simulink model "TMS_20260330_1321"  (R2024b)
settings: Solver=VariableStepAuto  StartTime=0.0  StopTime=10.0  RelTol=1e-3
settings Model: Creator=uiv53217  LastModifiedBy=uiv53217

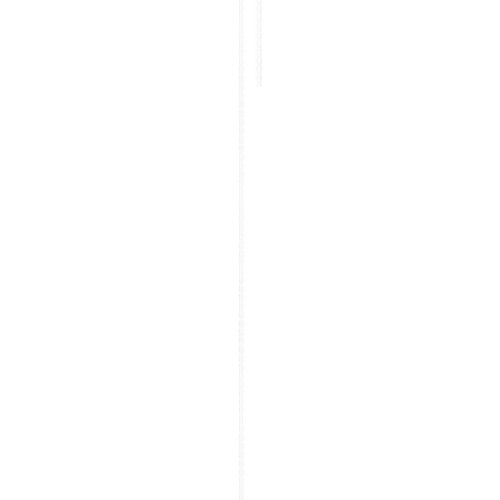
[thumbnail: Simulink's stored preview of the top-level diagram]
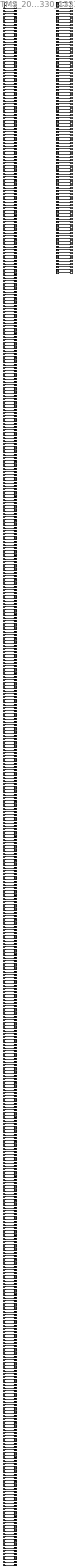
== system TMS_20260330_1321 ==
  OnOffReq_FL : Inport  OutDataTypeStr=uint8
  OnOffReq_FR : Inport  Port=2  OutDataTypeStr=uint8
  OnOffReq_RL : Inport  Port=3  OutDataTypeStr=uint8
  AutoReq_FL : Inport  Port=4  OutDataTypeStr=uint8
  AutoReq_FR : Inport  Port=5  OutDataTypeStr=uint8
  AutoReq_RL : Inport  Port=6  OutDataTypeStr=uint8
  MaxDefReq : Inport  Port=7  OutDataTypeStr=uint8
  FastVent : Inport  Port=8  OutDataTypeStr=uint8
  MaxACReq : Inport  Port=9  OutDataTypeStr=uint8
  MaxHeatReq : Inport  Port=10  OutDataTypeStr=uint8
  SmartClearReq : Inport  Port=11  OutDataTypeStr=uint8
  ACReq_FL : Inport  Port=12  OutDataTypeStr=uint8
  ACReq_FR : Inport  Port=13  OutDataTypeStr=uint8
  ACReq_RL : Inport  Port=14  OutDataTypeStr=uint8
  HeatReq_FL : Inport  Port=15  OutDataTypeStr=uint8
  HeatReq_FR : Inport  Port=16  OutDataTypeStr=uint8
  HeatReq_RL : Inport  Port=17  OutDataTypeStr=uint8
  VentReq_FL : Inport  Port=18  OutDataTypeStr=uint8
  VentReq_FR : Inport  Port=19  OutDataTypeStr=uint8
  VentReq_RL : Inport  Port=20  OutDataTypeStr=uint8
  TSet_FL : Inport  Port=21  OutDataTypeStr=uint16
  TSet_FR : Inport  Port=22  OutDataTypeStr=uint16
  TSet_RL : Inport  Port=23  OutDataTypeStr=uint16
  WindLvl_FL : Inport  Port=24  OutDataTypeStr=uint8
  WindLvl_FR : Inport  Port=25  OutDataTypeStr=uint8
  WindLvl_RL : Inport  Port=26  OutDataTypeStr=uint8
  OutletMode_FL : Inport  Port=27  OutDataTypeStr=uint8
  OutletMode_FR : Inport  Port=28  OutDataTypeStr=uint8
  OutletMode_RL : Inport  Port=29  OutDataTypeStr=uint8
  Sync : Inport  Port=30  OutDataTypeStr=uint8
  Inlet : Inport  Port=31  OutDataTypeStr=uint8
  ECO : Inport  Port=32  OutDataTypeStr=uint8
  AQS : Inport  Port=33  OutDataTypeStr=uint8
  RrWndHet : Inport  Port=34  OutDataTypeStr=uint8
  CfgAutoWindLvl : Inport  Port=35  OutDataTypeStr=uint8
  ACFrtPnlLckRrPnl : Inport  Port=36  OutDataTypeStr=uint8
  OccupantStsFL : Inport  Port=37  OutDataTypeStr=uint8
  OccupantStsFR : Inport  Port=38  OutDataTypeStr=uint8
  OccupantStsRL : Inport  Port=39  OutDataTypeStr=uint8
  OccupantStsRM : Inport  Port=40  OutDataTypeStr=uint8
  OccupantStsRR : Inport  Port=41  OutDataTypeStr=uint8
  CmptmtFrntWindDewT : Inport  Port=42  OutDataTypeStr=uint16
  CmptmtFrntWindT : Inport  Port=43  OutDataTypeStr=uint16
  CmptmtRelHum : Inport  Port=44  OutDataTypeStr=uint16
  RiSolarData : Inport  Port=45  OutDataTypeStr=uint8
  LeSolarData : Inport  Port=46  OutDataTypeStr=uint8
  VehSpd : Inport  Port=47  OutDataTypeStr=uint16
  CarModSts : Inport  Port=48  OutDataTypeStr=uint8
  UsgModSts : Inport  Port=49  OutDataTypeStr=uint8
  Cal_Sig_AmbTEna : Inport  Port=50  OutDataTypeStr=uint8
  Cal_Sig_AmbT : Inport  Port=51  OutDataTypeStr=uint16
  Cal_Sig_InCarTEna : Inport  Port=52  OutDataTypeStr=uint8
  Cal_Sig_InCarT : Inport  Port=53  OutDataTypeStr=uint16
  Cal_Sig_HvacEvaprTFrntEna : Inport  Port=54  OutDataTypeStr=uint8
  Cal_Sig_HvacEvaprTFrntT : Inport  Port=55  OutDataTypeStr=uint16
  Cal_Sig_HvacEvaprTReEna : Inport  Port=56  OutDataTypeStr=uint8
  Cal_Sig_HvacEvaprTReT : Inport  Port=57  OutDataTypeStr=uint16
  Cal_Sig_HvacCondsorTFrntTEna : Inport  Port=58  OutDataTypeStr=uint8
  Cal_Sig_HvacCondsorTFrntT : Inport  Port=59  OutDataTypeStr=uint16
  Cal_Sig_CooltT1Ena : Inport  Port=60  OutDataTypeStr=uint8
  Cal_Sig_CooltT1 : Inport  Port=61  OutDataTypeStr=uint16
  Cal_Sig_CooltT2Ena : Inport  Port=62  OutDataTypeStr=uint8
  Cal_Sig_CooltT2 : Inport  Port=63  OutDataTypeStr=uint16
  Cal_Sig_CooltT3Ena : Inport  Port=64  OutDataTypeStr=uint8
  Cal_Sig_CooltT3 : Inport  Port=65  OutDataTypeStr=uint16
  AutoDeHumPopUp : Inport  Port=66  OutDataTypeStr=uint8
  AutoDefrstPopUp : Inport  Port=67  OutDataTypeStr=uint8
  AutoFreshPopUp : Inport  Port=68  OutDataTypeStr=uint8
  ClimaDefrstSts : Inport  Port=69  OutDataTypeStr=uint8
  ClimaDefrstMaxSts : Inport  Port=70  OutDataTypeStr=uint8
  HvacFrntBlowerSts : Inport  Port=71  OutDataTypeStr=uint8
  HvacReBlowerSts : Inport  Port=72  OutDataTypeStr=uint8
  HvacAirMFlwFrntEstimd : Inport  Port=73  OutDataTypeStr=uint16
  HvacAirMFlwReEstimd : Inport  Port=74  OutDataTypeStr=uint16
  HvacAirQFlwFrntEstimd : Inport  Port=75  OutDataTypeStr=uint16
  HvacAirQFlwReEstimd : Inport  Port=76  OutDataTypeStr=uint16
  HvacFrntBlwSpdFb : Inport  Port=77  OutDataTypeStr=uint16
  HvacReBlwSpdFb : Inport  Port=78  OutDataTypeStr=uint16
  HvacCoolgEnaFrnt : Inport  Port=79  OutDataTypeStr=uint8
  HvacCoolgEnaRe : Inport  Port=80  OutDataTypeStr=uint8
  HvacDefrstFlapActlPosn : Inport  Port=81  OutDataTypeStr=uint16
  HvacEvaprTSpFrnt : Inport  Port=82  OutDataTypeStr=uint16
  HvacEvaprTSpRe : Inport  Port=83  OutDataTypeStr=uint16
  HvacModFlapActlPosnFrstRowLe : Inport  Port=84  OutDataTypeStr=uint16
  HvacModFlapActlPosnFrstRowRi : Inport  Port=85  OutDataTypeStr=uint16
  HvacModFlapActlPosnSecRowLe : Inport  Port=86  OutDataTypeStr=uint16
  HvacModFlapActlPosnSecRowRi : Inport  Port=87  OutDataTypeStr=uint16
  HvacOsaFlapActlPosn : Inport  Port=88  OutDataTypeStr=uint16
  HvacRecFlapActlPosn : Inport  Port=89  OutDataTypeStr=uint16
  HvacRecircActRat : Inport  Port=90  OutDataTypeStr=uint8
  HvacTempFlapActlPosnFrstRowLe : Inport  Port=91  OutDataTypeStr=uint16
  HvacTempFlapActlPosnFrstRowRi : Inport  Port=92  OutDataTypeStr=uint16
  HvacTempFlapActlPosnSecRowLe : Inport  Port=93  OutDataTypeStr=uint16
  HvacTempFlapActlPosnSecRowRi : Inport  Port=94  OutDataTypeStr=uint16
  HvacTgtAirTForRowFirstLe : Inport  Port=95  OutDataTypeStr=uint16
  HvacTgtAirTForRowFirstRi : Inport  Port=96  OutDataTypeStr=uint16
  HvacTgtAirTForRowSecLe : Inport  Port=97  OutDataTypeStr=uint16
  HvacTgtAirTForRowSecRi : Inport  Port=98  OutDataTypeStr=uint16
  AmbTEstimdAmbTEstimd : Inport  Port=99  OutDataTypeStr=uint16
  AmbTEstimdQf : Inport  Port=100  OutDataTypeStr=uint8
  CmptmtTFrntCmptmtTFrnt : Inport  Port=101  OutDataTypeStr=uint16
  CmptmtTFrntFanForCmptmtTRunng : Inport  Port=102  OutDataTypeStr=uint8
  CmptmtTFrntQf : Inport  Port=103  OutDataTypeStr=uint8
  CmptmtTReCmptmtTFrnt : Inport  Port=104  OutDataTypeStr=uint16
  CmptmtTReCmptmtTFrntQf : Inport  Port=105  OutDataTypeStr=uint8
  CmptmtTReFanForCmptmtTRunng : Inport  Port=106  OutDataTypeStr=uint8
  HvacEvaprTFrntTHvac : Inport  Port=107  OutDataTypeStr=uint16
  HvacEvaprTFrntTQf : Inport  Port=108  OutDataTypeStr=uint8
  HvacEvaprTReTHvac : Inport  Port=109  OutDataTypeStr=uint16
  HvacEvaprTReTQf : Inport  Port=110  OutDataTypeStr=uint8
  HvacAirTForRowFirstAtFlrLeTHvac : Inport  Port=111  OutDataTypeStr=uint16
  HvacAirTForRowFirstAtFlrLeTQf : Inport  Port=112  OutDataTypeStr=uint8
  HvacAirTForRowFirstAtFlrRiTHvac : Inport  Port=113  OutDataTypeStr=uint16
  HvacAirTForRowFirstAtFlrRiTQf : Inport  Port=114  OutDataTypeStr=uint8
  HvacAirTForRowFirstAtFaceLeTHvac : Inport  Port=115  OutDataTypeStr=uint16
  HvacAirTForRowFirstAtFaceLeTQf : Inport  Port=116  OutDataTypeStr=uint8
  HvacAirTForRowFirstAtFaceRiTHvac : Inport  Port=117  OutDataTypeStr=uint16
  HvacAirTForRowFirstAtFaceRiTQf : Inport  Port=118  OutDataTypeStr=uint8
  HvacAirTForRowSecAtFlrLeTHvac : Inport  Port=119  OutDataTypeStr=uint16
  HvacAirTForRowSecAtFlrLeTQf : Inport  Port=120  OutDataTypeStr=uint8
  HvacAirTForRowSecAtFlrRiTHvac : Inport  Port=121  OutDataTypeStr=uint16
  HvacAirTForRowSecAtFlrRiTQf : Inport  Port=122  OutDataTypeStr=uint8
  HvacAirTForRowSecAtFaceLeTHvac : Inport  Port=123  OutDataTypeStr=uint16
  HvacAirTForRowSecAtFaceLeTQf : Inport  Port=124  OutDataTypeStr=uint8
  HvacAirTForRowSecAtFaceRiTHvac : Inport  Port=125  OutDataTypeStr=uint16
  HvacAirTForRowSecAtFaceRiTQf : Inport  Port=126  OutDataTypeStr=uint8
  HvacCondsorTFrntTHvac : Inport  Port=127  OutDataTypeStr=uint16
  HvacCondsorTFrntTQf : Inport  Port=128  OutDataTypeStr=uint8
  HvacCondsorTspFrntTHvac : Inport  Port=129  OutDataTypeStr=uint16
  ClimaThermReq : Inport  Port=130  OutDataTypeStr=uint8
  ClimaThermSts : Inport  Port=131  OutDataTypeStr=uint8
  HvacAirTHvacIntkT : Inport  Port=132  OutDataTypeStr=uint16
  RsvdSigForClima01 : Inport  Port=133  OutDataTypeStr=uint8
  RsvdSigForClima02 : Inport  Port=134  OutDataTypeStr=uint8
  RsvdSigForClima03 : Inport  Port=135  OutDataTypeStr=uint8
  RsvdSigForClima04 : Inport  Port=136  OutDataTypeStr=uint8
  RsvdSigForClima05 : Inport  Port=137  OutDataTypeStr=uint8
  RsvdSigForClima06 : Inport  Port=138  OutDataTypeStr=uint8
  RsvdSigForClima07 : Inport  Port=139  OutDataTypeStr=uint8
  RsvdSigForClima08 : Inport  Port=140  OutDataTypeStr=uint8
  RsvdSigForClima09 : Inport  Port=141  OutDataTypeStr=uint8
  RsvdSigForClima10 : Inport  Port=142  OutDataTypeStr=uint8
  RsvdSigForClima11 : Inport  Port=143  OutDataTypeStr=uint8
  RsvdSigForClima12 : Inport  Port=144  OutDataTypeStr=uint8
  RsvdSigForClima13 : Inport  Port=145  OutDataTypeStr=uint8
  RsvdSigForClima14 : Inport  Port=146  OutDataTypeStr=uint8
  RsvdSigForClima15 : Inport  Port=147  OutDataTypeStr=uint8
  RsvdSigForClima16 : Inport  Port=148  OutDataTypeStr=uint8
  RsvdSigForClima17 : Inport  Port=149  OutDataTypeStr=uint8
  RsvdSigForClima18 : Inport  Port=150  OutDataTypeStr=uint8
  RsvdSigForClima19 : Inport  Port=151  OutDataTypeStr=uint8
  RsvdSigForClima20 : Inport  Port=152  OutDataTypeStr=uint8
  RsvdSigForClima21 : Inport  Port=153  OutDataTypeStr=uint8
  RsvdSigForClima22 : Inport  Port=154  OutDataTypeStr=uint8
  RsvdSigForClima23 : Inport  Port=155  OutDataTypeStr=uint8
  HvacDefrstFlapTgtPosn : Inport  Port=156  OutDataTypeStr=uint16
  HvacModFlapTgtPosnFrstRowLe : Inport  Port=157  OutDataTypeStr=uint16
  HvacModFlapTgtPosnFrstRowRi : Inport  Port=158  OutDataTypeStr=uint16
  HvacModFlapTgtPosnSecRowLe : Inport  Port=159  OutDataTypeStr=uint16
  HvacModFlapTgtPosnSecRowRi : Inport  Port=160  OutDataTypeStr=uint16
  HvacOsaFlapTgtPosn : Inport  Port=161  OutDataTypeStr=uint16
  HvacRecFlapTgtPosn : Inport  Port=162  OutDataTypeStr=uint16
  HvacTempFlapTgtPosnFrstRowLe : Inport  Port=163  OutDataTypeStr=uint16
  HvacTempFlapTgtPosnFrstRowRi : Inport  Port=164  OutDataTypeStr=uint16
  HvacTempFlapTgtPosnSecRowLe : Inport  Port=165  OutDataTypeStr=uint16
  HvacTempFlapTgtPosnSecRowRi : Inport  Port=166  OutDataTypeStr=uint16
  HvBattThermRunAway : Inport  Port=167  OutDataTypeStr=uint8
  WhlMotCooltFlowMinReq : Inport  Port=168  OutDataTypeStr=uint16
  WhlMotSysCoolgReq : Inport  Port=169  OutDataTypeStr=uint8
  WhlMotSysCooltT : Inport  Port=170  OutDataTypeStr=uint16
  WhlMotSysInvrT : Inport  Port=171  OutDataTypeStr=uint16
  WhlMotSysMotT : Inport  Port=172  OutDataTypeStr=uint16
  DCChrgSt : Inport  Port=173  OutDataTypeStr=uint8
  DCChrgnHndlSts : Inport  Port=174  OutDataTypeStr=uint8
  ACChrgSt : Inport  Port=175  OutDataTypeStr=uint8
  ACChrgnHndlSts : Inport  Port=176  OutDataTypeStr=uint8
  HvBattCooltFlowReq : Inport  Port=177  OutDataTypeStr=uint16
  HvBattCooltMaxTReq : Inport  Port=178  OutDataTypeStr=uint16
  HvBattCooltMinTReq : Inport  Port=179  OutDataTypeStr=uint16
  HvBattCooltTReq : Inport  Port=180  OutDataTypeStr=uint16
  HvBattThermReq : Inport  Port=181  OutDataTypeStr=uint8
  HvBattTAvg : Inport  Port=182  OutDataTypeStr=uint16
  HvBattTMax : Inport  Port=183  OutDataTypeStr=uint16
  HvBattTMin : Inport  Port=184  OutDataTypeStr=uint16
  HvBattActSOC : Inport  Port=185  OutDataTypeStr=uint16
  HvSysRlyStsChks : Inport  Port=186  OutDataTypeStr=uint8
  HvSysRlyStsCntr : Inport  Port=187  OutDataTypeStr=uint8
  HvSysRlyStsHvSysRlySts : Inport  Port=188  OutDataTypeStr=uint8
  HvCmprPwrAllwd : Inport  Port=189  OutDataTypeStr=uint8
  HvHeatrPwrAllwd : Inport  Port=190  OutDataTypeStr=uint8
  WhlMotCooltFlwEstimd : Inport  Port=191  OutDataTypeStr=uint16
  HvBattCooltFlwEstimd : Inport  Port=192  OutDataTypeStr=uint16
  HvBattThermReqFb : Inport  Port=193  OutDataTypeStr=uint8
  HvCmprNormPwrDes : Inport  Port=194  OutDataTypeStr=uint8
  HvHeatrNormPwrDes : Inport  Port=195  OutDataTypeStr=uint8
  HvCmprCritPwrDes : Inport  Port=196  OutDataTypeStr=uint8
  HvHeatrCritPwrDes : Inport  Port=197  OutDataTypeStr=uint8
  ThermDeiceReq : Inport  Port=198  OutDataTypeStr=uint8
  ThermRfgModReq : Inport  Port=199  OutDataTypeStr=uint8
  ThermRfgModSts : Inport  Port=200  OutDataTypeStr=uint8
  ThermRfgModSwtSts : Inport  Port=201  OutDataTypeStr=uint8
  ThermCooltModReq : Inport  Port=202  OutDataTypeStr=uint8
  ThermCooltModSts : Inport  Port=203  OutDataTypeStr=uint8
  ThermCooltModSwtSts : Inport  Port=204  OutDataTypeStr=uint8
  RfgSnsrT1 : Inport  Port=205  OutDataTypeStr=uint16
  RfgSnsrT2 : Inport  Port=206  OutDataTypeStr=uint16
  RfgSnsrT3 : Inport  Port=207  OutDataTypeStr=uint16
  RfgSnsrT4 : Inport  Port=208  OutDataTypeStr=uint16
  RfgSnsrP1 : Inport  Port=209  OutDataTypeStr=uint16
  RfgSnsrPT1T : Inport  Port=210  OutDataTypeStr=uint16
  RfgSnsrPT1P : Inport  Port=211  OutDataTypeStr=uint16
  RfgSnsrT5Rsvd : Inport  Port=212  OutDataTypeStr=uint16
  RfgSnsrT6Rsvd : Inport  Port=213  OutDataTypeStr=uint16
  RfgSnsrT7Rsvd : Inport  Port=214  OutDataTypeStr=uint16
  RfgSnsrT8Rsvd : Inport  Port=215  OutDataTypeStr=uint16
  RfgSnsrP5Rsvd : Inport  Port=216  OutDataTypeStr=uint16
  RfgSnsrP6Rsvd : Inport  Port=217  OutDataTypeStr=uint16
  RfgSnsrP7Rsvd : Inport  Port=218  OutDataTypeStr=uint16
  RfgSnsrP8Rsvd : Inport  Port=219  OutDataTypeStr=uint16
  CooltSnsrT1 : Inport  Port=220  OutDataTypeStr=uint16
  CooltSnsrT2 : Inport  Port=221  OutDataTypeStr=uint16
  CooltSnsrT3 : Inport  Port=222  OutDataTypeStr=uint16
  CooltSnsrT4Rsvd : Inport  Port=223  OutDataTypeStr=uint16
  CooltSnsrT5Rsvd : Inport  Port=224  OutDataTypeStr=uint16
  CooltSnsrT6Rsvd : Inport  Port=225  OutDataTypeStr=uint16
  CooltSnsrT7Rsvd : Inport  Port=226  OutDataTypeStr=uint16
  CooltSnsrT8Rsvd : Inport  Port=227  OutDataTypeStr=uint16
  CRFMAirMFlwEstimd : Inport  Port=228  OutDataTypeStr=uint16
  CRFMAirQFlwEstimd : Inport  Port=229  OutDataTypeStr=uint16
  ThermCptsSts : Inport  Port=230  OutDataTypeStr=uint32
  ThermProtnSts : Inport  Port=231  OutDataTypeStr=uint32
  ThermSysSts : Inport  Port=232  OutDataTypeStr=uint8
  RsvdSigForTherm01 : Inport  Port=233  OutDataTypeStr=uint8
  RsvdSigForTherm02 : Inport  Port=234  OutDataTypeStr=uint8
  RsvdSigForTherm03 : Inport  Port=235  OutDataTypeStr=uint8
  RsvdSigForTherm04 : Inport  Port=236  OutDataTypeStr=uint8
  RsvdSigForTherm05 : Inport  Port=237  OutDataTypeStr=uint8
  RsvdSigForTherm06 : Inport  Port=238  OutDataTypeStr=uint8
  RsvdSigForTherm07 : Inport  Port=239  OutDataTypeStr=uint8
  RsvdSigForTherm08 : Inport  Port=240  OutDataTypeStr=uint8
  RsvdSigForTherm09 : Inport  Port=241  OutDataTypeStr=uint8
  RsvdSigForTherm10 : Inport  Port=242  OutDataTypeStr=uint8
  RsvdSigForTherm11 : Inport  Port=243  OutDataTypeStr=uint8
  RsvdSigForTherm12 : Inport  Port=244  OutDataTypeStr=uint8
  RsvdSigForTherm13 : Inport  Port=245  OutDataTypeStr=uint8
  RsvdSigForTherm14 : Inport  Port=246  OutDataTypeStr=uint8
  RsvdSigForTherm15 : Inport  Port=247  OutDataTypeStr=uint8
  RsvdSigForTherm16 : Inport  Port=248  OutDataTypeStr=uint8
  RsvdSigForTherm17 : Inport  Port=249  OutDataTypeStr=uint8
  RsvdSigForTherm18 : Inport  Port=250  OutDataTypeStr=uint8
  RsvdSigForTherm19 : Inport  Port=251  OutDataTypeStr=uint8
  RsvdSigForTherm20 : Inport  Port=252  OutDataTypeStr=uint8
  RsvdSigForTherm21 : Inport  Port=253  OutDataTypeStr=uint8
  RsvdSigForTherm22 : Inport  Port=254  OutDataTypeStr=uint8
  RsvdSigForTherm23 : Inport  Port=255  OutDataTypeStr=uint8
  HeatrPmpPwmCmd : Inport  Port=256  OutDataTypeStr=uint16
  HvBattPmpPwmCmd : Inport  Port=257  OutDataTypeStr=uint16
  EldtPmpPwmCmd : Inport  Port=258  OutDataTypeStr=uint16
  SOV1OnOffCmd : Inport  Port=259  OutDataTypeStr=uint8
  SOV2OnOffCmd : Inport  Port=260  OutDataTypeStr=uint8
  SOV3OnOffCmd : Inport  Port=261  OutDataTypeStr=uint8
  CoolgFanPWMCmd : Inport  Port=262  OutDataTypeStr=uint16
  FrntBlwPWMCmd : Inport  Port=263  OutDataTypeStr=uint16
  BcfvNVMFlt : Inport  Port=264  OutDataTypeStr=uint8
  BctvNVMFlt : Inport  Port=265  OutDataTypeStr=uint8
  CmprEEPROMFault : Inport  Port=266  OutDataTypeStr=uint8
  CmprHVoltResonanceStat : Inport  Port=267  OutDataTypeStr=uint8
  CmprInCurrOverCurrStat : Inport  Port=268  OutDataTypeStr=uint8
  CmprLiquidSluggingStat : Inport  Port=269  OutDataTypeStr=uint8
  CmprLostCommStat : Inport  Port=270  OutDataTypeStr=uint8
  CmprMotorCurrOverCurrStat : Inport  Port=271  OutDataTypeStr=uint8
  CmprOverMotorCurrStat : Inport  Port=272  OutDataTypeStr=uint8
  CmprOverPowerStat : Inport  Port=273  OutDataTypeStr=uint8
  CmprRAMFault : Inport  Port=274  OutDataTypeStr=uint8
  CmprROMFault : Inport  Port=275  OutDataTypeStr=uint8
  CmprReqCmprPwrLim : Inport  Port=276  OutDataTypeStr=uint8
  CmprReqCmprRunReq : Inport  Port=277  OutDataTypeStr=uint8
  CmprReqCmprSpdReq : Inport  Port=278  OutDataTypeStr=uint8
  CmprRotorLockStat : Inport  Port=279  OutDataTypeStr=uint8
  CmprSpdIncrReq : Inport  Port=280  OutDataTypeStr=uint8
  CooltFlowInCmptmtCirc : Inport  Port=281  OutDataTypeStr=uint16
  HpBattFwvActvSaveReq : Inport  Port=282  OutDataTypeStr=uint8
  HpBattFwvFltSts : Inport  Port=283  OutDataTypeStr=uint8
  HpBattFwvMode : Inport  Port=284  OutDataTypeStr=uint8
  HpBattFwvPosRec : Inport  Port=285  OutDataTypeStr=uint16
  HpBattFwvPosSetReq : Inport  Port=286  OutDataTypeStr=uint8
  HpBattFwvRefDrvReq : Inport  Port=287  OutDataTypeStr=uint8
  HpBattFwvRunSts : Inport  Port=288  OutDataTypeStr=uint8
  HpBattFwvSpdLvl : Inport  Port=289  OutDataTypeStr=uint8
  HpBattFwvSpdLvlReq : Inport  Port=290  OutDataTypeStr=uint8
  HpBattFwvTempSts : Inport  Port=291  OutDataTypeStr=uint8
  HpBattFwvVoltSts : Inport  Port=292  OutDataTypeStr=uint8
  HpBattVlvActvSaveReq : Inport  Port=293  OutDataTypeStr=uint8
  HpBattVlvFltSts : Inport  Port=294  OutDataTypeStr=uint8
  HpBattVlvMode : Inport  Port=295  OutDataTypeStr=uint8
  HpBattVlvPosRec : Inport  Port=296  OutDataTypeStr=uint16
  HpBattVlvPosSetReq : Inport  Port=297  OutDataTypeStr=uint8
  HpBattVlvRefDrvReq : Inport  Port=298  OutDataTypeStr=uint8
  HpBattVlvRunSts : Inport  Port=299  OutDataTypeStr=uint8
  HpBattVlvSpdLvl : Inport  Port=300  OutDataTypeStr=uint8
  HpBattVlvSpdLvlReq : Inport  Port=301  OutDataTypeStr=uint8
  HpBattVlvTempSts : Inport  Port=302  OutDataTypeStr=uint8
  HpBattVlvVoltSts : Inport  Port=303  OutDataTypeStr=uint8
  HvCooltHeatrEnad : Inport  Port=304  OutDataTypeStr=uint8
  HvCooltHeatrICnsSig : Inport  Port=305  OutDataTypeStr=uint8
  HvCooltHeatrInfoCompProtn : Inport  Port=306  OutDataTypeStr=uint8
  HvCooltHeatrSplyUForCtrlUnitValSig : Inport  Port=307  OutDataTypeStr=uint8
  HvCooltHeatrStsSig : Inport  Port=308  OutDataTypeStr=uint8
  HvCooltWtrHeatrWtrTInIntk : Inport  Port=309  OutDataTypeStr=uint8
  HvCooltWtrHeatrWtrTInOutl : Inport  Port=310  OutDataTypeStr=uint8
  HvHeatrPwrCns : Inport  Port=311  OutDataTypeStr=uint16
  HvHeatrPwrCnsDes : Inport  Port=312  OutDataTypeStr=uint16
  HvWtrHeatrPwrCnsAllwd : Inport  Port=313  OutDataTypeStr=uint8
  HvWtrHeatrWtrTDes : Inport  Port=314  OutDataTypeStr=uint8
  CmprDiagcFbCmprCmprSpdErr : Inport  Port=315  OutDataTypeStr=uint8
  CmprDiagcFbCmprCtrlrErr : Inport  Port=316  OutDataTypeStr=uint8
  CmprDiagcFbCmprDrvrCircSnsr : Inport  Port=317  OutDataTypeStr=uint8
  CmprDiagcFbCmprDrvrCircSnsrPlaus : Inport  Port=318  OutDataTypeStr=uint8
  CmprDiagcFbCmprHvSnsr1 : Inport  Port=319  OutDataTypeStr=uint8
  CmprDiagcFbCmprHvSnsr2 : Inport  Port=320  OutDataTypeStr=uint8
  CmprDiagcFbCmprHvSnsrI : Inport  Port=321  OutDataTypeStr=uint8
  CmprDiagcFbCmprHvSnsrICrct : Inport  Port=322  OutDataTypeStr=uint8
  CmprDiagcFbCmprHvSnsrIPlaus : Inport  Port=323  OutDataTypeStr=uint8
  CmprDiagcFbCmprHvSnsrPlaus : Inport  Port=324  OutDataTypeStr=uint8
  CmprDiagcFbCmprHvSplyErr : Inport  Port=325  OutDataTypeStr=uint8
  CmprDiagcFbCmprPhaseWire : Inport  Port=326  OutDataTypeStr=uint8
  CmprDiagcFbCmprT1 : Inport  Port=327  OutDataTypeStr=uint8
  CmprDiagcFbCmprT2 : Inport  Port=328  OutDataTypeStr=uint8
  CmprDiagcFbCmprTOperErr1 : Inport  Port=329  OutDataTypeStr=uint8
  CmprDiagcFbCmprTOperErr2 : Inport  Port=330  OutDataTypeStr=uint8
  CmprDiagcFbCmprTPlaus : Inport  Port=331  OutDataTypeStr=uint8
  CmprDiagcFbCmprUSplyErr : Inport  Port=332  OutDataTypeStr=uint8
  CmprFbCmprI : Inport  Port=333  OutDataTypeStr=uint16
  CmprFbCmprIPha : Inport  Port=334  OutDataTypeStr=uint8
  CmprFbCmprSpd : Inport  Port=335  OutDataTypeStr=uint8
  CmprFbCmprSts1 : Inport  Port=336  OutDataTypeStr=uint8
  CmprFbCmprSts2 : Inport  Port=337  OutDataTypeStr=uint8
  CmprFbCmprT1 : Inport  Port=338  OutDataTypeStr=uint8
  CmprFbCmprT2 : Inport  Port=339  OutDataTypeStr=uint8
  CmprFbCmprU : Inport  Port=340  OutDataTypeStr=uint16
  EctvCmdVlvMovEna : Inport  Port=341  OutDataTypeStr=uint8
  EctvCmdVlvPosSetReq : Inport  Port=342  OutDataTypeStr=uint8
  EctvCmdVlvSpdLvlReq : Inport  Port=343  OutDataTypeStr=uint8
  EctvStatVlvFaultSts : Inport  Port=344  OutDataTypeStr=uint8
  EctvStatVlvPosSts : Inport  Port=345  OutDataTypeStr=uint8
  EctvStatVlvRunSts : Inport  Port=346  OutDataTypeStr=uint8
  EctvStatVlvSpdLvl : Inport  Port=347  OutDataTypeStr=uint8
  EctvStatVlvTempSts : Inport  Port=348  OutDataTypeStr=uint8
  EctvStatVoltSts : Inport  Port=349  OutDataTypeStr=uint8
  HvCooltHeatrEnadWhE2EChks : Inport  Port=350  OutDataTypeStr=uint8
  HvCooltHeatrEnadWhE2ECntr : Inport  Port=351  OutDataTypeStr=uint8
  HvCooltHeatrEnadWhE2EHvchEnad : Inport  Port=352  OutDataTypeStr=uint8
  HvCooltHeatrProtnOfSelfTmpSigHwProtn : Inport  Port=353  OutDataTypeStr=uint8
  HvCooltHeatrProtnOfSelfTmpSigOvrheatg : Inport  Port=354  OutDataTypeStr=uint8
  HvCooltHeatrProtnOfSelfTmpSigProtnOfSelfTmp : Inport  Port=355  OutDataTypeStr=uint8
  HvCooltHeatrProtnOfSelfTmpSigProtnOfSelfTmpResd : Inport  Port=356  OutDataTypeStr=uint8
  HvCooltHeatrSnsrFltSigCooltTInSnsrFlt : Inport  Port=357  OutDataTypeStr=uint8
  HvCooltHeatrSnsrFltSigCooltTOutSnsrFlt : Inport  Port=358  OutDataTypeStr=uint8
  HvCooltHeatrSnsrFltSigResdForSnsrFlt : Inport  Port=359  OutDataTypeStr=uint8
  HvCooltHeatrSnsrFltSigTInMtrlSnsrFlt : Inport  Port=360  OutDataTypeStr=uint8
  HvCooltHeatrSrvRqrdSigCircForDrvrShoOrOpen : Inport  Port=361  OutDataTypeStr=uint8
  HvCooltHeatrSrvRqrdSigICnsOutOfRng : Inport  Port=362  OutDataTypeStr=uint8
  HvCooltHeatrSrvRqrdSigMemErr : Inport  Port=363  OutDataTypeStr=uint8
  HvCooltHeatrSrvRqrdSigSrvRqrd : Inport  Port=364  OutDataTypeStr=uint8
  HvCooltHeatrSrvRqrdSigSrvRqrdResd : Inport  Port=365  OutDataTypeStr=uint8
  HvCooltHeatrStsWhE2EChks : Inport  Port=366  OutDataTypeStr=uint8
  HvCooltHeatrStsWhE2ECntr : Inport  Port=367  OutDataTypeStr=uint8
  HvCooltHeatrStsWhE2EHvchSts : Inport  Port=368  OutDataTypeStr=uint8
  HvCooltHeatrWarnSigCooltTOutOfRng : Inport  Port=369  OutDataTypeStr=uint8
  HvCooltHeatrWarnSigFltInCom : Inport  Port=370  OutDataTypeStr=uint8
  HvCooltHeatrWarnSigFltPrsnt : Inport  Port=371  OutDataTypeStr=uint8
  HvCooltHeatrWarnSigFltPrsntResd : Inport  Port=372  OutDataTypeStr=uint8
  HvCooltHeatrWarnSigHvOutOfRng : Inport  Port=373  OutDataTypeStr=uint8
  HvCooltHeatrWarnSigULoOutOfRng : Inport  Port=374  OutDataTypeStr=uint8
  BexvNVMFlt : Inport  Port=375  OutDataTypeStr=uint8
  CexvNVMFlt : Inport  Port=376  OutDataTypeStr=uint8
  EexvNVMFlt : Inport  Port=377  OutDataTypeStr=uint8
  BexvPosnReqExvCalibReq : Inport  Port=378  OutDataTypeStr=uint8
  BexvPosnReqExvHeatdReq : Inport  Port=379  OutDataTypeStr=uint8
  BexvPosnReqExvMovEnable : Inport  Port=380  OutDataTypeStr=uint8
  BexvPosnReqExvPosnReq : Inport  Port=381  OutDataTypeStr=uint16
  BexvStsExvActrPosn : Inport  Port=382  OutDataTypeStr=uint16
  BexvStsExvBlkErr : Inport  Port=383  OutDataTypeStr=uint8
  BexvStsExvCalibSts : Inport  Port=384  OutDataTypeStr=uint8
  BexvStsExvElecStsErr : Inport  Port=385  OutDataTypeStr=uint8
  BexvStsExvMovSts : Inport  Port=386  OutDataTypeStr=uint8
  BexvStsExvOvrTempErr : Inport  Port=387  OutDataTypeStr=uint8
  BexvStsExvOvrTrvlErr : Inport  Port=388  OutDataTypeStr=uint8
  BexvStsExvPreHeatgSts : Inport  Port=389  OutDataTypeStr=uint8
  BexvStsExvVoltgRangErr : Inport  Port=390  OutDataTypeStr=uint8
  CexvPosnReqExvCalibReq : Inport  Port=391  OutDataTypeStr=uint8
  CexvPosnReqExvHeatdReq : Inport  Port=392  OutDataTypeStr=uint8
  CexvPosnReqExvMovEnable : Inport  Port=393  OutDataTypeStr=uint8
  CexvPosnReqExvPosnReq : Inport  Port=394  OutDataTypeStr=uint16
  CexvStsExvActrPosn : Inport  Port=395  OutDataTypeStr=uint16
  CexvStsExvBlkErr : Inport  Port=396  OutDataTypeStr=uint8
  CexvStsExvCalibSts : Inport  Port=397  OutDataTypeStr=uint8
  CexvStsExvElecStsErr : Inport  Port=398  OutDataTypeStr=uint8
  CexvStsExvMovSts : Inport  Port=399  OutDataTypeStr=uint8
  CexvStsExvOvrTempErr : Inport  Port=400  OutDataTypeStr=uint8
  CexvStsExvOvrTrvlErr : Inport  Port=401  OutDataTypeStr=uint8
  CexvStsExvPreHeatgSts : Inport  Port=402  OutDataTypeStr=uint8
  CexvStsExvVoltgRangErr : Inport  Port=403  OutDataTypeStr=uint8
  EexvPosnReqExvCalibReq : Inport  Port=404  OutDataTypeStr=uint8
  EexvPosnReqExvHeatdReq : Inport  Port=405  OutDataTypeStr=uint8
  EexvPosnReqExvMovEnable : Inport  Port=406  OutDataTypeStr=uint8
  EexvPosnReqExvPosnReq : Inport  Port=407  OutDataTypeStr=uint16
  EexvStsExvActrPosn : Inport  Port=408  OutDataTypeStr=uint16
  EexvStsExvBlkErr : Inport  Port=409  OutDataTypeStr=uint8
  EexvStsExvCalibSts : Inport  Port=410  OutDataTypeStr=uint8
  EexvStsExvElecStsErr : Inport  Port=411  OutDataTypeStr=uint8
  EexvStsExvMovSts : Inport  Port=412  OutDataTypeStr=uint8
  EexvStsExvOvrTempErr : Inport  Port=413  OutDataTypeStr=uint8
  EexvStsExvOvrTrvlErr : Inport  Port=414  OutDataTypeStr=uint8
  EexvStsExvPreHeatgSts : Inport  Port=415  OutDataTypeStr=uint8
  EexvStsExvVoltgRangErr : Inport  Port=416  OutDataTypeStr=uint8
  AGMNVMFlt : Inport  Port=417  OutDataTypeStr=uint8
  GrlActTrqBoost : Inport  Port=418  OutDataTypeStr=uint8
  GrlAutoCalibReq : Inport  Port=419  OutDataTypeStr=uint8
  GrlHldTrqActive : Inport  Port=420  OutDataTypeStr=uint8
  GrlShttrMoveActive : Inport  Port=421  OutDataTypeStr=uint8
  GrlShttrOverVolt : Inport  Port=422  OutDataTypeStr=uint8
  GrlShttrOvertravelErr : Inport  Port=423  OutDataTypeStr=uint8
  GrlTrqBoostReq : Inport  Port=424  OutDataTypeStr=uint8
  GrlShttrDmdShttrCalEna : Inport  Port=425  OutDataTypeStr=uint8
  GrlShttrDmdShttrPosnReq : Inport  Port=426  OutDataTypeStr=uint8
  GrlShttrStsShttrActrFlt : Inport  Port=427  OutDataTypeStr=uint8
  GrlShttrStsShttrBlkd : Inport  Port=428  OutDataTypeStr=uint8
  GrlShttrStsShttrCalActv : Inport  Port=429  OutDataTypeStr=uint8
  GrlShttrStsShttrCalIndcd : Inport  Port=430  OutDataTypeStr=uint8
  GrlShttrStsShttrElecErr : Inport  Port=431  OutDataTypeStr=uint8
  GrlShttrStsShttrPosnRaw : Inport  Port=432  OutDataTypeStr=uint8
  GrlShttrStsShttrSnsrFlt : Inport  Port=433  OutDataTypeStr=uint8
  GrlShttrStsShttrTErr : Inport  Port=434  OutDataTypeStr=uint8
  GrlShttrStsShttrULoErr : Inport  Port=435  OutDataTypeStr=uint8
  AFUGenErr : Inport  Port=436  OutDataTypeStr=uint8
  AirFragActEnad : Inport  Port=437  OutDataTypeStr=uint8
  AirFragCh1 : Inport  Port=438  OutDataTypeStr=uint8
  AirFragCh1AvlTi : Inport  Port=439  OutDataTypeStr=uint16
  AirFragCh1RunngSts : Inport  Port=440  OutDataTypeStr=uint8
  AirFragCh1Type : Inport  Port=441  OutDataTypeStr=uint8
  AirFragCh2 : Inport  Port=442  OutDataTypeStr=uint8
  AirFragCh2AvlTi : Inport  Port=443  OutDataTypeStr=uint16
  AirFragCh2RunngSts : Inport  Port=444  OutDataTypeStr=uint8
  AirFragCh2Type : Inport  Port=445  OutDataTypeStr=uint8
  AirFragCh3 : Inport  Port=446  OutDataTypeStr=uint8
  AirFragCh3AvlTi : Inport  Port=447  OutDataTypeStr=uint16
  AirFragCh3RunngSts : Inport  Port=448  OutDataTypeStr=uint8
  AirFragCh3Type : Inport  Port=449  OutDataTypeStr=uint8
  AirFragCh4 : Inport  Port=450  OutDataTypeStr=uint8
  AirFragCh4AvlTi : Inport  Port=451  OutDataTypeStr=uint16
  AirFragCh4RunngSts : Inport  Port=452  OutDataTypeStr=uint8
  AirFragCh4Type : Inport  Port=453  OutDataTypeStr=uint8
  AirFragCh5 : Inport  Port=454  OutDataTypeStr=uint8
  AirFragCh5AvlTi : Inport  Port=455  OutDataTypeStr=uint16
  AirFragCh5RunngSts : Inport  Port=456  OutDataTypeStr=uint8
  AirFragCh5Type : Inport  Port=457  OutDataTypeStr=uint8
  AirFragChgSts : Inport  Port=458  OutDataTypeStr=uint8
  AirFragConcReq : Inport  Port=459  OutDataTypeStr=uint8
  AirFragFanErr : Inport  Port=460  OutDataTypeStr=uint8
  AirFragInitSts : Inport  Port=461  OutDataTypeStr=uint8
  AirFragLvlRspn : Inport  Port=462  OutDataTypeStr=uint8
  AirFragMot1Err : Inport  Port=463  OutDataTypeStr=uint8
  AirFragMot2Err : Inport  Port=464  OutDataTypeStr=uint8
  AirFragMot3Err : Inport  Port=465  OutDataTypeStr=uint8
  AirFragMot4Err : Inport  Port=466  OutDataTypeStr=uint8
  AirFragMot5Err : Inport  Port=467  OutDataTypeStr=uint8
  AirFragOvrVoltErr : Inport  Port=468  OutDataTypeStr=uint8
  AirFragTempErr : Inport  Port=469  OutDataTypeStr=uint8
  AirFragUndVoltErr : Inport  Port=470  OutDataTypeStr=uint8
  CmpmtInAirPmAQI : Inport  Port=471  OutDataTypeStr=uint8
  CmpmtInAirPmDnsty : Inport  Port=472  OutDataTypeStr=uint16
  HvacAirMFlowVent : Inport  Port=473  OutDataTypeStr=uint16
  HvacRecircAct : Inport  Port=474  OutDataTypeStr=uint8
  InPm25FanErr : Inport  Port=475  OutDataTypeStr=uint8
  InPm25SensrIntErr : Inport  Port=476  OutDataTypeStr=uint8
  InPm25SnrTempErr : Inport  Port=477  OutDataTypeStr=uint8
  InPm25SnrVoltgRangErr : Inport  Port=478  OutDataTypeStr=uint8
  InPm25SnsrActnReq : Inport  Port=479  OutDataTypeStr=uint8
  InPm25SnsrElecErr : Inport  Port=480  OutDataTypeStr=uint8
  InPm25SnsrSts : Inport  Port=481  OutDataTypeStr=uint8
  CmptmtAirTEstimdExtdComptmtT : Inport  Port=482  OutDataTypeStr=uint16
  CmptmtAirTEstimdExtdQlyFlg : Inport  Port=483  OutDataTypeStr=uint8
  VehMktForPmSnsrAirMtrlSnsrReq : Inport  Port=484  OutDataTypeStr=uint8
  VehMktForPmSnsrVehMktGlb : Inport  Port=485  OutDataTypeStr=uint8
  IoRx_FrntBlwPwmFlt_u8 : Inport  Port=486  OutDataTypeStr=uint8
  IoRx_FrntBlwFrqFb_u16 : Inport  Port=487  OutDataTypeStr=uint16
  IoRx_DCMot1ActVoltRaw_u16 : Inport  Port=488  OutDataTypeStr=uint16
  IoRx_DCMot2ActVoltRaw_u16 : Inport  Port=489  OutDataTypeStr=uint16
  IoRx_DCMot3ActVoltRaw_u16 : Inport  Port=490  OutDataTypeStr=uint16
  IoRx_DCMot4ActVoltRaw_u16 : Inport  Port=491  OutDataTypeStr=uint16
  IoRx_DCMot5ActVoltRaw_u16 : Inport  Port=492  OutDataTypeStr=uint16
  IoRx_DCMot6ActVoltRaw_u16 : Inport  Port=493  OutDataTypeStr=uint16
  IoRx_DCMot7ActVoltRaw_u16 : Inport  Port=494  OutDataTypeStr=uint16
  IoRx_DCMot1HbrFltFb_u8 : Inport  Port=495  OutDataTypeStr=uint8
  IoRx_DCMot2HbrFltFb_u8 : Inport  Port=496  OutDataTypeStr=uint8
  IoRx_DCMot3HbrFltFb_u8 : Inport  Port=497  OutDataTypeStr=uint8
  IoRx_DCMot4HbrFltFb_u8 : Inport  Port=498  OutDataTypeStr=uint8
  IoRx_DCMot5HbrFltFb_u8 : Inport  Port=499  OutDataTypeStr=uint8
  IoRx_DCMot6HbrFltFb_u8 : Inport  Port=500  OutDataTypeStr=uint8
  IoRx_DCMot7HbrFltFb_u8 : Inport  Port=501  OutDataTypeStr=uint8
  IoRx_FrntCbnTVoltRaw_u16 : Inport  Port=502  OutDataTypeStr=uint16
  IoRx_FrntHexTVoltRaw_u16 : Inport  Port=503  OutDataTypeStr=uint16
  IoRx_FrntEvapTVoltRaw_u16 : Inport  Port=504  OutDataTypeStr=uint16
  IoRx_FrntLeFaceTVoltRaw_u16 : Inport  Port=505  OutDataTypeStr=uint16
  IoRx_FrntLeFootTVoltRaw_u16 : Inport  Port=506  OutDataTypeStr=uint16
  IoRx_FrntRiFaceTVoltRaw_u16 : Inport  Port=507  OutDataTypeStr=uint16
  IoRx_FrntRiFootTVoltRaw_u16 : Inport  Port=508  OutDataTypeStr=uint16
  IoRx_ReLeFaceTVoltRaw_u16 : Inport  Port=509  OutDataTypeStr=uint16
  IoRx_ReLeFootTVoltRaw_u16 : Inport  Port=510  OutDataTypeStr=uint16
  IoRx_AmbTVoltRaw_u16 : Inport  Port=511  OutDataTypeStr=uint16
  IoRx_EnvtAQSPwmFb_u16 : Inport  Port=512  OutDataTypeStr=uint16
  IoRx_FrntCbnTFanRlyFlt_u8 : Inport  Port=513  OutDataTypeStr=uint8
  IoRx_ClimtRlyFlt_u8 : Inport  Port=514  OutDataTypeStr=uint8
  IoRx_ClimtPwrRlyFlt_u8 : Inport  Port=515  OutDataTypeStr=uint8
  IoRx_HvBattPmpPwmFlt_u8 : Inport  Port=516  OutDataTypeStr=uint8
  IoRx_EldtPmpPwmFlt_u8 : Inport  Port=517  OutDataTypeStr=uint8
  IoRx_HeatrPmpPwmFlt_u8 : Inport  Port=518  OutDataTypeStr=uint8
  IoRx_CoolgFanPwmFlt_u8 : Inport  Port=519  OutDataTypeStr=uint8
  IoRx_SOV1RlyFlt_u8 : Inport  Port=520  OutDataTypeStr=uint8
  IoRx_SOV2RlyFlt_u8 : Inport  Port=521  OutDataTypeStr=uint8
  IoRx_SOV3RlyFlt_u8 : Inport  Port=522  OutDataTypeStr=uint8
  IoRx_RfgP1VoltRaw_u16 : Inport  Port=523  OutDataTypeStr=uint16
  IoRx_RfgT1VoltRaw_u16 : Inport  Port=524  OutDataTypeStr=uint16
  IoRx_RfgT2VoltRaw_u16 : Inport  Port=525  OutDataTypeStr=uint16
  IoRx_RfgT3VoltRaw_u16 : Inport  Port=526  OutDataTypeStr=uint16
  IoRx_RfgT4VoltRaw_u16 : Inport  Port=527  OutDataTypeStr=uint16
  IoRx_RfgPT1PVoltRaw_u16 : Inport  Port=528  OutDataTypeStr=uint16
  IoRx_RfgPT1TVoltRaw_u16 : Inport  Port=529  OutDataTypeStr=uint16
  IoRx_CooltT1VoltRaw_u16 : Inport  Port=530  OutDataTypeStr=uint16
  IoRx_CooltT2VoltRaw_u16 : Inport  Port=531  OutDataTypeStr=uint16
  IoRx_CooltT3VoltRaw_u16 : Inport  Port=532  OutDataTypeStr=uint16
  IoRx_CooltT4VoltRaw_u16 : Inport  Port=533  OutDataTypeStr=uint16
  IoRx_ThermPwr1RlyFlt_u8 : Inport  Port=534  OutDataTypeStr=uint8
  IoRx_ThermPwr2RlyFlt_u8 : Inport  Port=535  OutDataTypeStr=uint8
  IoRx_ThermPwr3RlyFlt_u8 : Inport  Port=536  OutDataTypeStr=uint8
  IoRx_CoolgFanRlyFlt_u8 : Inport  Port=537  OutDataTypeStr=uint8
  IoRx_PmpRlyFlt_u8 : Inport  Port=538  OutDataTypeStr=uint8
  RcpR_AmbTRawR : Inport  Port=539  OutDataTypeStr=uint8
  RcpR_RfgT1RawR : Inport  Port=540  OutDataTypeStr=uint8
  RcpR_RfgT2RawR : Inport  Port=541  OutDataTypeStr=uint8
  RcpR_RfgT3RawR : Inport  Port=542  OutDataTypeStr=uint8
  RcpR_RfgT4RawR : Inport  Port=543  OutDataTypeStr=uint8
  RcpR_RfgPT1TRawR : Inport  Port=544  OutDataTypeStr=uint8
  RcpR_CooltT1RawR : Inport  Port=545  OutDataTypeStr=uint8
  RcpR_CooltT2RawR : Inport  Port=546  OutDataTypeStr=uint8
  RcpR_CooltT3RawR : Inport  Port=547  OutDataTypeStr=uint8
  RcpR_CooltT4RawR : Inport  Port=548  OutDataTypeStr=uint8
  RcpR_FrntCbnTRawR : Inport  Port=549  OutDataTypeStr=uint8
  RcpR_FrntHexTRawR : Inport  Port=550  OutDataTypeStr=uint8
  RcpR_FrntEvapTRawR : Inport  Port=551  OutDataTypeStr=uint8
  RcpR_FrntLeFaceTRawR : Inport  Port=552  OutDataTypeStr=uint8
  RcpR_FrntLeFootTRawR : Inport  Port=553  OutDataTypeStr=uint8
  RcpR_FrntRiFaceTRawR : Inport  Port=554  OutDataTypeStr=uint8
  RcpR_FrntRiFootTRawR : Inport  Port=555  OutDataTypeStr=uint8
  RcpR_ReLeFaceTRawR : Inport  Port=556  OutDataTypeStr=uint8
  RcpR_ReLeFootTRawR : Inport  Port=557  OutDataTypeStr=uint8
  ACChrgSt_Terminator : Terminator
  ACChrgnHndlSts_Terminator : Terminator
  ACFrtPnlLckRrPnl_Terminator : Terminator
  ACReq_FL_Terminator : Terminator
  ACReq_FR_Terminator : Terminator
  ACReq_RL_Terminator : Terminator
  AFUGenErr_Terminator : Terminator
  AGMNVMFlt_Terminator : Terminator
  AQS_Terminator : Terminator
  AirFragActEnad_Terminator : Terminator
  AirFragCh1AvlTi_Terminator : Terminator
  AirFragCh1RunngSts_Terminator : Terminator
  AirFragCh1Type_Terminator : Terminator
  AirFragCh1_Terminator : Terminator
  AirFragCh2AvlTi_Terminator : Terminator
  AirFragCh2RunngSts_Terminator : Terminator
  AirFragCh2Type_Terminator : Terminator
  AirFragCh2_Terminator : Terminator
  AirFragCh3AvlTi_Terminator : Terminator
  AirFragCh3RunngSts_Terminator : Terminator
  AirFragCh3Type_Terminator : Terminator
  AirFragCh3_Terminator : Terminator
  AirFragCh4AvlTi_Terminator : Terminator
  AirFragCh4RunngSts_Terminator : Terminator
  AirFragCh4Type_Terminator : Terminator
  AirFragCh4_Terminator : Terminator
  AirFragCh5AvlTi_Terminator : Terminator
  AirFragCh5RunngSts_Terminator : Terminator
  AirFragCh5Type_Terminator : Terminator
  AirFragCh5_Terminator : Terminator
  AirFragChgSts_Terminator : Terminator
  AirFragConcReq_Terminator : Terminator
  AirFragFanErr_Terminator : Terminator
  AirFragInitSts_Terminator : Terminator
  AirFragLvlRspn_Terminator : Terminator
  AirFragMot1Err_Terminator : Terminator
  AirFragMot2Err_Terminator : Terminator
  AirFragMot3Err_Terminator : Terminator
  AirFragMot4Err_Terminator : Terminator
  AirFragMot5Err_Terminator : Terminator
  AirFragOvrVoltErr_Terminator : Terminator
  AirFragTempErr_Terminator : Terminator
  AirFragUndVoltErr_Terminator : Terminator
  AmbTEstimdAmbTEstimd_Terminator : Terminator
  AmbTEstimdQf_Terminator : Terminator
  AutoDeHumPopUp_Terminator : Terminator
  AutoDefrstPopUp_Terminator : Terminator
  AutoFreshPopUp_Terminator : Terminator
  AutoReq_FL_Terminator : Terminator
  AutoReq_FR_Terminator : Terminator
  AutoReq_RL_Terminator : Terminator
  BcfvNVMFlt_Terminator : Terminator
  BctvNVMFlt_Terminator : Terminator
  BexvNVMFlt_Terminator : Terminator
  BexvPosnReqExvCalibReq_Terminator : Terminator
  BexvPosnReqExvHeatdReq_Terminator : Terminator
  BexvPosnReqExvMovEnable_Terminator : Terminator
  BexvPosnReqExvPosnReq_Terminator : Terminator
  BexvStsExvActrPosn_Terminator : Terminator
  BexvStsExvBlkErr_Terminator : Terminator
  BexvStsExvCalibSts_Terminator : Terminator
  BexvStsExvElecStsErr_Terminator : Terminator
  BexvStsExvMovSts_Terminator : Terminator
  BexvStsExvOvrTempErr_Terminator : Terminator
  BexvStsExvOvrTrvlErr_Terminator : Terminator
  BexvStsExvPreHeatgSts_Terminator : Terminator
  BexvStsExvVoltgRangErr_Terminator : Terminator
  CRFMAirMFlwEstimd_Terminator : Terminator
  CRFMAirQFlwEstimd_Terminator : Terminator
  Cal_Sig_AmbTEna_Terminator : Terminator
  Cal_Sig_AmbT_Terminator : Terminator
  Cal_Sig_CooltT1Ena_Terminator : Terminator
  Cal_Sig_CooltT1_Terminator : Terminator
  Cal_Sig_CooltT2Ena_Terminator : Terminator
  Cal_Sig_CooltT2_Terminator : Terminator
  Cal_Sig_CooltT3Ena_Terminator : Terminator
  Cal_Sig_CooltT3_Terminator : Terminator
  Cal_Sig_HvacCondsorTFrntTEna_Terminator : Terminator
  Cal_Sig_HvacCondsorTFrntT_Terminator : Terminator
  Cal_Sig_HvacEvaprTFrntEna_Terminator : Terminator
  Cal_Sig_HvacEvaprTFrntT_Terminator : Terminator
  Cal_Sig_HvacEvaprTReEna_Terminator : Terminator
  Cal_Sig_HvacEvaprTReT_Terminator : Terminator
  Cal_Sig_InCarTEna_Terminator : Terminator
  Cal_Sig_InCarT_Terminator : Terminator
  CarModSts_Terminator : Terminator
  CexvNVMFlt_Terminator : Terminator
  CexvPosnReqExvCalibReq_Terminator : Terminator
  CexvPosnReqExvHeatdReq_Terminator : Terminator
  CexvPosnReqExvMovEnable_Terminator : Terminator
  CexvPosnReqExvPosnReq_Terminator : Terminator
  CexvStsExvActrPosn_Terminator : Terminator
  CexvStsExvBlkErr_Terminator : Terminator
  CexvStsExvCalibSts_Terminator : Terminator
  CexvStsExvElecStsErr_Terminator : Terminator
  CexvStsExvMovSts_Terminator : Terminator
  CexvStsExvOvrTempErr_Terminator : Terminator
  CexvStsExvOvrTrvlErr_Terminator : Terminator
  CexvStsExvPreHeatgSts_Terminator : Terminator
  CexvStsExvVoltgRangErr_Terminator : Terminator
  CfgAutoWindLvl_Terminator : Terminator
  ClimaDefrstMaxSts_Terminator : Terminator
  ClimaDefrstSts_Terminator : Terminator
  ClimaThermReq_Terminator : Terminator
  ClimaThermSts_Terminator : Terminator
  CmpmtInAirPmAQI_Terminator : Terminator
  CmpmtInAirPmDnsty_Terminator : Terminator
  CmprDiagcFbCmprCmprSpdErr_Terminator : Terminator
  CmprDiagcFbCmprCtrlrErr_Terminator : Terminator
  CmprDiagcFbCmprDrvrCircSnsrPlaus_Terminator : Terminator
  CmprDiagcFbCmprDrvrCircSnsr_Terminator : Terminator
  CmprDiagcFbCmprHvSnsr1_Terminator : Terminator
  CmprDiagcFbCmprHvSnsr2_Terminator : Terminator
  CmprDiagcFbCmprHvSnsrICrct_Terminator : Terminator
  CmprDiagcFbCmprHvSnsrIPlaus_Terminator : Terminator
  CmprDiagcFbCmprHvSnsrI_Terminator : Terminator
  CmprDiagcFbCmprHvSnsrPlaus_Terminator : Terminator
  CmprDiagcFbCmprHvSplyErr_Terminator : Terminator
  CmprDiagcFbCmprPhaseWire_Terminator : Terminator
  CmprDiagcFbCmprT1_Terminator : Terminator
  CmprDiagcFbCmprT2_Terminator : Terminator
  CmprDiagcFbCmprTOperErr1_Terminator : Terminator
  CmprDiagcFbCmprTOperErr2_Terminator : Terminator
  CmprDiagcFbCmprTPlaus_Terminator : Terminator
  CmprDiagcFbCmprUSplyErr_Terminator : Terminator
  CmprEEPROMFault_Terminator : Terminator
  CmprFbCmprIPha_Terminator : Terminator
  CmprFbCmprI_Terminator : Terminator
  CmprFbCmprSpd_Terminator : Terminator
  CmprFbCmprSts1_Terminator : Terminator
  CmprFbCmprSts2_Terminator : Terminator
  CmprFbCmprT1_Terminator : Terminator
  CmprFbCmprT2_Terminator : Terminator
  CmprFbCmprU_Terminator : Terminator
  CmprHVoltResonanceStat_Terminator : Terminator
  CmprInCurrOverCurrStat_Terminator : Terminator
  CmprLiquidSluggingStat_Terminator : Terminator
  CmprLostCommStat_Terminator : Terminator
  CmprMotorCurrOverCurrStat_Terminator : Terminator
  CmprOverMotorCurrStat_Terminator : Terminator
  CmprOverPowerStat_Terminator : Terminator
  CmprRAMFault_Terminator : Terminator
  CmprROMFault_Terminator : Terminator
  CmprReqCmprPwrLim_Terminator : Terminator
  CmprReqCmprRunReq_Terminator : Terminator
  CmprReqCmprSpdReq_Terminator : Terminator
  CmprRotorLockStat_Terminator : Terminator
  CmprSpdIncrReq_Terminator : Terminator
  CmptmtAirTEstimdExtdComptmtT_Terminator : Terminator
  CmptmtAirTEstimdExtdQlyFlg_Terminator : Terminator
  CmptmtFrntWindDewT_Terminator : Terminator
  CmptmtFrntWindT_Terminator : Terminator
  CmptmtRelHum_Terminator : Terminator
  CmptmtTFrntCmptmtTFrnt_Terminator : Terminator
  CmptmtTFrntFanForCmptmtTRunng_Terminator : Terminator
  CmptmtTFrntQf_Terminator : Terminator
  CmptmtTReCmptmtTFrntQf_Terminator : Terminator
  CmptmtTReCmptmtTFrnt_Terminator : Terminator
  CmptmtTReFanForCmptmtTRunng_Terminator : Terminator
  CoolgFanPWMCmd_Terminator : Terminator
  CooltFlowInCmptmtCirc_Terminator : Terminator
  CooltSnsrT1_Terminator : Terminator
  CooltSnsrT2_Terminator : Terminator
  CooltSnsrT3_Terminator : Terminator
  CooltSnsrT4Rsvd_Terminator : Terminator
  CooltSnsrT5Rsvd_Terminator : Terminator
  CooltSnsrT6Rsvd_Terminator : Terminator
  CooltSnsrT7Rsvd_Terminator : Terminator
  CooltSnsrT8Rsvd_Terminator : Terminator
  DCChrgSt_Terminator : Terminator
  DCChrgnHndlSts_Terminator : Terminator
  ECO_Terminator : Terminator
  EctvCmdVlvMovEna_Terminator : Terminator
  EctvCmdVlvPosSetReq_Terminator : Terminator
  EctvCmdVlvSpdLvlReq_Terminator : Terminator
  EctvStatVlvFaultSts_Terminator : Terminator
  EctvStatVlvPosSts_Terminator : Terminator
  EctvStatVlvRunSts_Terminator : Terminator
  EctvStatVlvSpdLvl_Terminator : Terminator
  EctvStatVlvTempSts_Terminator : Terminator
  EctvStatVoltSts_Terminator : Terminator
  EexvNVMFlt_Terminator : Terminator
  EexvPosnReqExvCalibReq_Terminator : Terminator
  EexvPosnReqExvHeatdReq_Terminator : Terminator
  EexvPosnReqExvMovEnable_Terminator : Terminator
  EexvPosnReqExvPosnReq_Terminator : Terminator
  EexvStsExvActrPosn_Terminator : Terminator
  EexvStsExvBlkErr_Terminator : Terminator
  EexvStsExvCalibSts_Terminator : Terminator
  EexvStsExvElecStsErr_Terminator : Terminator
  EexvStsExvMovSts_Terminator : Terminator
  EexvStsExvOvrTempErr_Terminator : Terminator
  EexvStsExvOvrTrvlErr_Terminator : Terminator
  EexvStsExvPreHeatgSts_Terminator : Terminator
  EexvStsExvVoltgRangErr_Terminator : Terminator
  EldtPmpPwmCmd_Terminator : Terminator
  FastVent_Terminator : Terminator
  FrntBlwPWMCmd_Terminator : Terminator
  GrlActTrqBoost_Terminator : Terminator
  GrlAutoCalibReq_Terminator : Terminator
  GrlHldTrqActive_Terminator : Terminator
  GrlShttrDmdShttrCalEna_Terminator : Terminator
  GrlShttrDmdShttrPosnReq_Terminator : Terminator
  GrlShttrMoveActive_Terminator : Terminator
  GrlShttrOverVolt_Terminator : Terminator
  GrlShttrOvertravelErr_Terminator : Terminator
  GrlShttrStsShttrActrFlt_Terminator : Terminator
  GrlShttrStsShttrBlkd_Terminator : Terminator
  GrlShttrStsShttrCalActv_Terminator : Terminator
  GrlShttrStsShttrCalIndcd_Terminator : Terminator
  GrlShttrStsShttrElecErr_Terminator : Terminator
  GrlShttrStsShttrPosnRaw_Terminator : Terminator
  GrlShttrStsShttrSnsrFlt_Terminator : Terminator
  GrlShttrStsShttrTErr_Terminator : Terminator
  GrlShttrStsShttrULoErr_Terminator : Terminator
  GrlTrqBoostReq_Terminator : Terminator
  HMI_ACDsp_Fr_Ground : Ground
  HMI_ACDsp_Rr_Ground : Ground
  HMI_ACFrtPnlLckRrPnlDsp_Ground : Ground
  HMI_AC_Fr_Ground : Ground
  HMI_AC_Rr_Ground : Ground
  HMI_AQSDsp_Ground : Ground
  HMI_AQS_Ground : Ground
  HMI_AutoManuDsp_Fr_Ground : Ground
  HMI_AutoManuDsp_Rr_Ground : Ground
  HMI_CfgAutoWindLvlDsp_Ground : Ground
  HMI_CfgAutoWindLvl_Ground : Ground
  HMI_ECODsp_Ground : Ground
  HMI_ECO_Ground : Ground
  HMI_FastVentDsp_Ground : Ground
  HMI_HMIOnSts_Fr_Ground : Ground
  HMI_HMIOnSts_Rr_Ground : Ground
  HMI_HMISts_Fr_Ground : Ground
  HMI_HMISts_Rr_Ground : Ground
  HMI_HeatDsp_Fr_Ground : Ground
  HMI_HeatDsp_Rr_Ground : Ground
  HMI_Heat_Fr_Ground : Ground
  HMI_Heat_Rr_Ground : Ground
  HMI_InletDsp_Ground : Ground
  HMI_Inlet_Ground : Ground
  HMI_MaxACDsp_Fr_Ground : Ground
  HMI_MaxACDsp_Rr_Ground : Ground
  HMI_MaxDefDsp_Ground : Ground
  HMI_MaxHeatDsp_Fr_Ground : Ground
  HMI_MaxHeatDsp_Rr_Ground : Ground
  HMI_OnOffDsp_Fr_Ground : Ground
  HMI_OnOffDsp_Rr_Ground : Ground
  HMI_OutletModeDsp_Fr_Ground : Ground
  HMI_OutletModeDsp_Rr_Ground : Ground
  HMI_OutletMode_Fr_Ground : Ground
  HMI_OutletMode_Rr_Ground : Ground
  HMI_RrWndHetDsp_Ground : Ground
  HMI_RrWndHet_Ground : Ground
  HMI_SyncDsp_Ground : Ground
  HMI_Sync_Ground : Ground
  HMI_TSetDsp_FL_Ground : Ground
  HMI_TSetDsp_FR_Ground : Ground
  HMI_TSetDsp_Rr_Ground : Ground
  HMI_TSet_FL_Ground : Ground
  HMI_TSet_FR_Ground : Ground
  HMI_TSet_Rr_Ground : Ground
  HMI_VentDsp_Fr_Ground : Ground
  HMI_VentDsp_Rr_Ground : Ground
  HMI_Vent_Fr_Ground : Ground
  HMI_Vent_Rr_Ground : Ground
  HMI_WindLvlDsp_FL_Ground : Ground
  HMI_WindLvlDsp_FR_Ground : Ground
  HMI_WindLvlDsp_Rr_Ground : Ground
  HMI_WindLvl_FL_Ground : Ground
  HMI_WindLvl_FR_Ground : Ground
  HMI_WindLvl_Rr_Ground : Ground
  HeatReq_FL_Terminator : Terminator
  HeatReq_FR_Terminator : Terminator
  HeatReq_RL_Terminator : Terminator
  HeatrPmpPwmCmd_Terminator : Terminator
  HpBattFwvActvSaveReq_Terminator : Terminator
  HpBattFwvFltSts_Terminator : Terminator
  HpBattFwvMode_Terminator : Terminator
  HpBattFwvPosRec_Terminator : Terminator
  HpBattFwvPosSetReq_Terminator : Terminator
  HpBattFwvRefDrvReq_Terminator : Terminator
  HpBattFwvRunSts_Terminator : Terminator
  HpBattFwvSpdLvlReq_Terminator : Terminator
  HpBattFwvSpdLvl_Terminator : Terminator
  HpBattFwvTempSts_Terminator : Terminator
  HpBattFwvVoltSts_Terminator : Terminator
  HpBattVlvActvSaveReq_Terminator : Terminator
  HpBattVlvFltSts_Terminator : Terminator
  HpBattVlvMode_Terminator : Terminator
  HpBattVlvPosRec_Terminator : Terminator
  HpBattVlvPosSetReq_Terminator : Terminator
  HpBattVlvRefDrvReq_Terminator : Terminator
  HpBattVlvRunSts_Terminator : Terminator
  HpBattVlvSpdLvlReq_Terminator : Terminator
  HpBattVlvSpdLvl_Terminator : Terminator
  HpBattVlvTempSts_Terminator : Terminator
  HpBattVlvVoltSts_Terminator : Terminator
  HvBattActSOC_Terminator : Terminator
  HvBattCooltFlowReq_Terminator : Terminator
  HvBattCooltFlwEstimd_Terminator : Terminator
  HvBattCooltMaxTReq_Terminator : Terminator
  HvBattCooltMinTReq_Terminator : Terminator
  HvBattCooltTReq_Terminator : Terminator
  HvBattPmpPwmCmd_Terminator : Terminator
  HvBattTAvg_Terminator : Terminator
  HvBattTMax_Terminator : Terminator
  HvBattTMin_Terminator : Terminator
  HvBattThermReqFb_Terminator : Terminator
  HvBattThermReq_Terminator : Terminator
  HvBattThermRunAway_Terminator : Terminator
  HvCmprCritPwrDes_Terminator : Terminator
  HvCmprNormPwrDes_Terminator : Terminator
  HvCmprPwrAllwd_Terminator : Terminator
  HvCooltHeatrEnadWhE2EChks_Terminator : Terminator
  HvCooltHeatrEnadWhE2ECntr_Terminator : Terminator
  HvCooltHeatrEnadWhE2EHvchEnad_Terminator : Terminator
  HvCooltHeatrEnad_Terminator : Terminator
  HvCooltHeatrICnsSig_Terminator : Terminator
  HvCooltHeatrInfoCompProtn_Terminator : Terminator
  HvCooltHeatrProtnOfSelfTmpSigHwProtn_Terminator : Terminator
  HvCooltHeatrProtnOfSelfTmpSigOvrheatg_Terminator : Terminator
  HvCooltHeatrProtnOfSelfTmpSigProtnOfSelfTmpResd_Terminator : Terminator
  HvCooltHeatrProtnOfSelfTmpSigProtnOfSelfTmp_Terminator : Terminator
  HvCooltHeatrSnsrFltSigCooltTInSnsrFlt_Terminator : Terminator
  HvCooltHeatrSnsrFltSigCooltTOutSnsrFlt_Terminator : Terminator
  HvCooltHeatrSnsrFltSigResdForSnsrFlt_Terminator : Terminator
  HvCooltHeatrSnsrFltSigTInMtrlSnsrFlt_Terminator : Terminator
  HvCooltHeatrSplyUForCtrlUnitValSig_Terminator : Terminator
  HvCooltHeatrSrvRqrdSigCircForDrvrShoOrOpen_Terminator : Terminator
  HvCooltHeatrSrvRqrdSigICnsOutOfRng_Terminator : Terminator
  HvCooltHeatrSrvRqrdSigMemErr_Terminator : Terminator
  HvCooltHeatrSrvRqrdSigSrvRqrdResd_Terminator : Terminator
  HvCooltHeatrSrvRqrdSigSrvRqrd_Terminator : Terminator
  HvCooltHeatrStsSig_Terminator : Terminator
  HvCooltHeatrStsWhE2EChks_Terminator : Terminator
  HvCooltHeatrStsWhE2ECntr_Terminator : Terminator
  HvCooltHeatrStsWhE2EHvchSts_Terminator : Terminator
  HvCooltHeatrWarnSigCooltTOutOfRng_Terminator : Terminator
  HvCooltHeatrWarnSigFltInCom_Terminator : Terminator
  HvCooltHeatrWarnSigFltPrsntResd_Terminator : Terminator
  HvCooltHeatrWarnSigFltPrsnt_Terminator : Terminator
  HvCooltHeatrWarnSigHvOutOfRng_Terminator : Terminator
  HvCooltHeatrWarnSigULoOutOfRng_Terminator : Terminator
  HvCooltWtrHeatrWtrTInIntk_Terminator : Terminator
  HvCooltWtrHeatrWtrTInOutl_Terminator : Terminator
  HvHeatrCritPwrDes_Terminator : Terminator
  HvHeatrNormPwrDes_Terminator : Terminator
  HvHeatrPwrAllwd_Terminator : Terminator
  HvHeatrPwrCnsDes_Terminator : Terminator
  HvHeatrPwrCns_Terminator : Terminator
  HvSysRlyStsChks_Terminator : Terminator
  HvSysRlyStsCntr_Terminator : Terminator
  HvSysRlyStsHvSysRlySts_Terminator : Terminator
  HvWtrHeatrPwrCnsAllwd_Terminator : Terminator
  HvWtrHeatrWtrTDes_Terminator : Terminator
  HvacAirMFlowVent_Terminator : Terminator
  HvacAirMFlwFrntEstimd_Terminator : Terminator
  HvacAirMFlwReEstimd_Terminator : Terminator
  HvacAirQFlwFrntEstimd_Terminator : Terminator
  HvacAirQFlwReEstimd_Terminator : Terminator
  HvacAirTForRowFirstAtFaceLeTHvac_Terminator : Terminator
  HvacAirTForRowFirstAtFaceLeTQf_Terminator : Terminator
  HvacAirTForRowFirstAtFaceRiTHvac_Terminator : Terminator
  HvacAirTForRowFirstAtFaceRiTQf_Terminator : Terminator
  HvacAirTForRowFirstAtFlrLeTHvac_Terminator : Terminator
  HvacAirTForRowFirstAtFlrLeTQf_Terminator : Terminator
  HvacAirTForRowFirstAtFlrRiTHvac_Terminator : Terminator
  HvacAirTForRowFirstAtFlrRiTQf_Terminator : Terminator
  HvacAirTForRowSecAtFaceLeTHvac_Terminator : Terminator
  HvacAirTForRowSecAtFaceLeTQf_Terminator : Terminator
  HvacAirTForRowSecAtFaceRiTHvac_Terminator : Terminator
  HvacAirTForRowSecAtFaceRiTQf_Terminator : Terminator
  HvacAirTForRowSecAtFlrLeTHvac_Terminator : Terminator
  HvacAirTForRowSecAtFlrLeTQf_Terminator : Terminator
  HvacAirTForRowSecAtFlrRiTHvac_Terminator : Terminator
  HvacAirTForRowSecAtFlrRiTQf_Terminator : Terminator
  HvacAirTHvacIntkT_Terminator : Terminator
  HvacCondsorTFrntTHvac_Terminator : Terminator
  HvacCondsorTFrntTQf_Terminator : Terminator
  HvacCondsorTspFrntTHvac_Terminator : Terminator
  HvacCoolgEnaFrnt_Terminator : Terminator
  HvacCoolgEnaRe_Terminator : Terminator
  HvacDefrstFlapActlPosn_Terminator : Terminator
  HvacDefrstFlapTgtPosn_Terminator : Terminator
  HvacEvaprTFrntTHvac_Terminator : Terminator
  HvacEvaprTFrntTQf_Terminator : Terminator
  HvacEvaprTReTHvac_Terminator : Terminator
  HvacEvaprTReTQf_Terminator : Terminator
  HvacEvaprTSpFrnt_Terminator : Terminator
  HvacEvaprTSpRe_Terminator : Terminator
  HvacFrntBlowerSts_Terminator : Terminator
  HvacFrntBlwSpdFb_Terminator : Terminator
  HvacModFlapActlPosnFrstRowLe_Terminator : Terminator
  HvacModFlapActlPosnFrstRowRi_Terminator : Terminator
  HvacModFlapActlPosnSecRowLe_Terminator : Terminator
  HvacModFlapActlPosnSecRowRi_Terminator : Terminator
  HvacModFlapTgtPosnFrstRowLe_Terminator : Terminator
  HvacModFlapTgtPosnFrstRowRi_Terminator : Terminator
  HvacModFlapTgtPosnSecRowLe_Terminator : Terminator
  HvacModFlapTgtPosnSecRowRi_Terminator : Terminator
  HvacOsaFlapActlPosn_Terminator : Terminator
  HvacOsaFlapTgtPosn_Terminator : Terminator
  HvacReBlowerSts_Terminator : Terminator
  HvacReBlwSpdFb_Terminator : Terminator
  HvacRecFlapActlPosn_Terminator : Terminator
  HvacRecFlapTgtPosn_Terminator : Terminator
  HvacRecircActRat_Terminator : Terminator
  HvacRecircAct_Terminator : Terminator
  HvacTempFlapActlPosnFrstRowLe_Terminator : Terminator
  HvacTempFlapActlPosnFrstRowRi_Terminator : Terminator
  HvacTempFlapActlPosnSecRowLe_Terminator : Terminator
  HvacTempFlapActlPosnSecRowRi_Terminator : Terminator
  HvacTempFlapTgtPosnFrstRowLe_Terminator : Terminator
  HvacTempFlapTgtPosnFrstRowRi_Terminator : Terminator
  HvacTempFlapTgtPosnSecRowLe_Terminator : Terminator
  HvacTempFlapTgtPosnSecRowRi_Terminator : Terminator
  HvacTgtAirTForRowFirstLe_Terminator : Terminator
  HvacTgtAirTForRowFirstRi_Terminator : Terminator
  HvacTgtAirTForRowSecLe_Terminator : Terminator
  HvacTgtAirTForRowSecRi_Terminator : Terminator
  InPm25FanErr_Terminator : Terminator
  InPm25SensrIntErr_Terminator : Terminator
  InPm25SnrTempErr_Terminator : Terminator
  InPm25SnrVoltgRangErr_Terminator : Terminator
  InPm25SnsrActnReq_Terminator : Terminator
  InPm25SnsrElecErr_Terminator : Terminator
  InPm25SnsrSts_Terminator : Terminator
  Inlet_Terminator : Terminator
  IoRx_AmbTVoltRaw_u16_Terminator : Terminator
  IoRx_ClimtPwrRlyFlt_u8_Terminator : Terminator
  IoRx_ClimtRlyFlt_u8_Terminator : Terminator
  IoRx_CoolgFanPwmFlt_u8_Terminator : Terminator
  IoRx_CoolgFanRlyFlt_u8_Terminator : Terminator
  IoRx_CooltT1VoltRaw_u16_Terminator : Terminator
  IoRx_CooltT2VoltRaw_u16_Terminator : Terminator
  IoRx_CooltT3VoltRaw_u16_Terminator : Terminator
  IoRx_CooltT4VoltRaw_u16_Terminator : Terminator
  IoRx_DCMot1ActVoltRaw_u16_Terminator : Terminator
  IoRx_DCMot1HbrFltFb_u8_Terminator : Terminator
  IoRx_DCMot2ActVoltRaw_u16_Terminator : Terminator
  IoRx_DCMot2HbrFltFb_u8_Terminator : Terminator
  IoRx_DCMot3ActVoltRaw_u16_Terminator : Terminator
  IoRx_DCMot3HbrFltFb_u8_Terminator : Terminator
  IoRx_DCMot4ActVoltRaw_u16_Terminator : Terminator
  IoRx_DCMot4HbrFltFb_u8_Terminator : Terminator
  IoRx_DCMot5ActVoltRaw_u16_Terminator : Terminator
  IoRx_DCMot5HbrFltFb_u8_Terminator : Terminator
  IoRx_DCMot6ActVoltRaw_u16_Terminator : Terminator
  IoRx_DCMot6HbrFltFb_u8_Terminator : Terminator
  IoRx_DCMot7ActVoltRaw_u16_Terminator : Terminator
  IoRx_DCMot7HbrFltFb_u8_Terminator : Terminator
  IoRx_EldtPmpPwmFlt_u8_Terminator : Terminator
  IoRx_EnvtAQSPwmFb_u16_Terminator : Terminator
  IoRx_FrntBlwFrqFb_u16_Terminator : Terminator
  IoRx_FrntBlwPwmFlt_u8_Terminator : Terminator
  IoRx_FrntCbnTFanRlyFlt_u8_Terminator : Terminator
  IoRx_FrntCbnTVoltRaw_u16_Terminator : Terminator
  IoRx_FrntEvapTVoltRaw_u16_Terminator : Terminator
  IoRx_FrntHexTVoltRaw_u16_Terminator : Terminator
  IoRx_FrntLeFaceTVoltRaw_u16_Terminator : Terminator
  IoRx_FrntLeFootTVoltRaw_u16_Terminator : Terminator
  IoRx_FrntRiFaceTVoltRaw_u16_Terminator : Terminator
  IoRx_FrntRiFootTVoltRaw_u16_Terminator : Terminator
  IoRx_HeatrPmpPwmFlt_u8_Terminator : Terminator
  IoRx_HvBattPmpPwmFlt_u8_Terminator : Terminator
  IoRx_PmpRlyFlt_u8_Terminator : Terminator
  IoRx_ReLeFaceTVoltRaw_u16_Terminator : Terminator
  IoRx_ReLeFootTVoltRaw_u16_Terminator : Terminator
  IoRx_RfgP1VoltRaw_u16_Terminator : Terminator
  IoRx_RfgPT1PVoltRaw_u16_Terminator : Terminator
  IoRx_RfgPT1TVoltRaw_u16_Terminator : Terminator
  IoRx_RfgT1VoltRaw_u16_Terminator : Terminator
  IoRx_RfgT2VoltRaw_u16_Terminator : Terminator
  IoRx_RfgT3VoltRaw_u16_Terminator : Terminator
  IoRx_RfgT4VoltRaw_u16_Terminator : Terminator
  IoRx_SOV1RlyFlt_u8_Terminator : Terminator
  IoRx_SOV2RlyFlt_u8_Terminator : Terminator
  IoRx_SOV3RlyFlt_u8_Terminator : Terminator
  IoRx_ThermPwr1RlyFlt_u8_Terminator : Terminator
  IoRx_ThermPwr2RlyFlt_u8_Terminator : Terminator
  IoRx_ThermPwr3RlyFlt_u8_Terminator : Terminator
  IoTx_ClimtPwrRly_b_Ground : Ground
  IoTx_ClimtRly_b_Ground : Ground
  IoTx_CoolgFanFrqCmd_u16_Ground : Ground
  IoTx_CoolgFanPwmCmd_u16_Ground : Ground
  IoTx_CoolgFanRly_b_Ground : Ground
  IoTx_DCMot1FrqCmd_u16_Ground : Ground
  IoTx_DCMot1PwmCmd_u16_Ground : Ground
  IoTx_DCMot1RunDir_u8_Ground : Ground
  IoTx_DCMot2FrqCmd_u16_Ground : Ground
  IoTx_DCMot2PwmCmd_u16_Ground : Ground
  IoTx_DCMot2RunDir_u8_Ground : Ground
  IoTx_DCMot3FrqCmd_u16_Ground : Ground
  IoTx_DCMot3PwmCmd_u16_Ground : Ground
  IoTx_DCMot3RunDir_u8_Ground : Ground
  IoTx_DCMot4FrqCmd_u16_Ground : Ground
  IoTx_DCMot4PwmCmd_u16_Ground : Ground
  IoTx_DCMot4RunDir_u8_Ground : Ground
  IoTx_DCMot5FrqCmd_u16_Ground : Ground
  IoTx_DCMot5PwmCmd_u16_Ground : Ground
  IoTx_DCMot5RunDir_u8_Ground : Ground
  IoTx_DCMot6FrqCmd_u16_Ground : Ground
  IoTx_DCMot6PwmCmd_u16_Ground : Ground
  IoTx_DCMot6RunDir_u8_Ground : Ground
  IoTx_DCMot7FrqCmd_u16_Ground : Ground
  IoTx_DCMot7PwmCmd_u16_Ground : Ground
  IoTx_DCMot7RunDir_u8_Ground : Ground
  IoTx_EldtPmpFrqCmd_u16_Ground : Ground
  IoTx_EldtPmpPwmCmd_u16_Ground : Ground
  IoTx_FrntBlwFrqCmd_u16_Ground : Ground
  IoTx_FrntBlwPwmCmd_u16_Ground : Ground
  IoTx_FrntCbnTFanRly_b_Ground : Ground
  IoTx_HeatrPmpFrqCmd_u16_Ground : Ground
  IoTx_HeatrPmpPwmCmd_u16_Ground : Ground
  IoTx_HvBattPmpFrqCmd_u16_Ground : Ground
  IoTx_HvBattPmpPwmCmd_u16_Ground : Ground
  IoTx_PmpRly_b_Ground : Ground
  IoTx_SOV1Rly_b_Ground : Ground
  IoTx_SOV2Rly_b_Ground : Ground
  IoTx_SOV3Rly_b_Ground : Ground
  IoTx_ThermPwr1Rly_b_Ground : Ground
  IoTx_ThermPwr2Rly_b_Ground : Ground
  IoTx_ThermPwr3Rly_b_Ground : Ground
  LeSolarData_Terminator : Terminator
  MaxACReq_Terminator : Terminator
  MaxDefReq_Terminator : Terminator
  MaxHeatReq_Terminator : Terminator
  OccupantStsFL_Terminator : Terminator
  OccupantStsFR_Terminator : Terminator
  OccupantStsRL_Terminator : Terminator
  OccupantStsRM_Terminator : Terminator
  OccupantStsRR_Terminator : Terminator
  OnOffReq_FL_Terminator : Terminator
  OnOffReq_FR_Terminator : Terminator
  OnOffReq_RL_Terminator : Terminator
  OutletMode_FL_Terminator : Terminator
  OutletMode_FR_Terminator : Terminator
  OutletMode_RL_Terminator : Terminator
  RcpR_AmbTRawR_Terminator : Terminator
  RcpR_CooltT1RawR_Terminator : Terminator
  RcpR_CooltT2RawR_Terminator : Terminator
  RcpR_CooltT3RawR_Terminator : Terminator
  RcpR_CooltT4RawR_Terminator : Terminator
  RcpR_FrntCbnTRawR_Terminator : Terminator
  RcpR_FrntEvapTRawR_Terminator : Terminator
  RcpR_FrntHexTRawR_Terminator : Terminator
  RcpR_FrntLeFaceTRawR_Terminator : Terminator
  RcpR_FrntLeFootTRawR_Terminator : Terminator
  RcpR_FrntRiFaceTRawR_Terminator : Terminator
  RcpR_FrntRiFootTRawR_Terminator : Terminator
  RcpR_ReLeFaceTRawR_Terminator : Terminator
  RcpR_ReLeFootTRawR_Terminator : Terminator
  RcpR_RfgPT1TRawR_Terminator : Terminator
  RcpR_RfgT1RawR_Terminator : Terminator
  RcpR_RfgT2RawR_Terminator : Terminator
  RcpR_RfgT3RawR_Terminator : Terminator
  RcpR_RfgT4RawR_Terminator : Terminator
  RfgSnsrP1_Terminator : Terminator
  RfgSnsrP5Rsvd_Terminator : Terminator
  RfgSnsrP6Rsvd_Terminator : Terminator
  RfgSnsrP7Rsvd_Terminator : Terminator
  RfgSnsrP8Rsvd_Terminator : Terminator
  RfgSnsrPT1P_Terminator : Terminator
  RfgSnsrPT1T_Terminator : Terminator
  RfgSnsrT1_Terminator : Terminator
  RfgSnsrT2_Terminator : Terminator
  RfgSnsrT3_Terminator : Terminator
  RfgSnsrT4_Terminator : Terminator
  RfgSnsrT5Rsvd_Terminator : Terminator
  RfgSnsrT6Rsvd_Terminator : Terminator
  RfgSnsrT7Rsvd_Terminator : Terminator
  RfgSnsrT8Rsvd_Terminator : Terminator
  RiSolarData_Terminator : Terminator
  RrWndHet_Terminator : Terminator
  RsvdSigForClima01_Terminator : Terminator
  RsvdSigForClima02_Terminator : Terminator
  RsvdSigForClima03_Terminator : Terminator
  RsvdSigForClima04_Terminator : Terminator
  RsvdSigForClima05_Terminator : Terminator
  RsvdSigForClima06_Terminator : Terminator
  RsvdSigForClima07_Terminator : Terminator
  RsvdSigForClima08_Terminator : Terminator
  RsvdSigForClima09_Terminator : Terminator
  RsvdSigForClima10_Terminator : Terminator
  RsvdSigForClima11_Terminator : Terminator
  RsvdSigForClima12_Terminator : Terminator
  RsvdSigForClima13_Terminator : Terminator
  RsvdSigForClima14_Terminator : Terminator
  RsvdSigForClima15_Terminator : Terminator
  RsvdSigForClima16_Terminator : Terminator
  RsvdSigForClima17_Terminator : Terminator
  RsvdSigForClima18_Terminator : Terminator
  RsvdSigForClima19_Terminator : Terminator
  RsvdSigForClima20_Terminator : Terminator
  RsvdSigForClima21_Terminator : Terminator
  RsvdSigForClima22_Terminator : Terminator
  RsvdSigForClima23_Terminator : Terminator
  RsvdSigForTherm01_Terminator : Terminator
  RsvdSigForTherm02_Terminator : Terminator
  RsvdSigForTherm03_Terminator : Terminator
  RsvdSigForTherm04_Terminator : Terminator
  RsvdSigForTherm05_Terminator : Terminator
  RsvdSigForTherm06_Terminator : Terminator
  RsvdSigForTherm07_Terminator : Terminator
  RsvdSigForTherm08_Terminator : Terminator
  RsvdSigForTherm09_Terminator : Terminator
  RsvdSigForTherm10_Terminator : Terminator
  RsvdSigForTherm11_Terminator : Terminator
  RsvdSigForTherm12_Terminator : Terminator
  RsvdSigForTherm13_Terminator : Terminator
  RsvdSigForTherm14_Terminator : Terminator
  RsvdSigForTherm15_Terminator : Terminator
  RsvdSigForTherm16_Terminator : Terminator
  RsvdSigForTherm17_Terminator : Terminator
  RsvdSigForTherm18_Terminator : Terminator
  RsvdSigForTherm19_Terminator : Terminator
  RsvdSigForTherm20_Terminator : Terminator
  RsvdSigForTherm21_Terminator : Terminator
  RsvdSigForTherm22_Terminator : Terminator
  RsvdSigForTherm23_Terminator : Terminator
  SOV1OnOffCmd_Terminator : Terminator
  SOV2OnOffCmd_Terminator : Terminator
  SOV3OnOffCmd_Terminator : Terminator
  SmartClearReq_Terminator : Terminator
  Sync_Terminator : Terminator
  TSet_FL_Terminator : Terminator
  TSet_FR_Terminator : Terminator
  TSet_RL_Terminator : Terminator
  ThermCooltModReq_Terminator : Terminator
  ThermCooltModSts_Terminator : Terminator
  ThermCooltModSwtSts_Terminator : Terminator
  ThermCptsSts_Terminator : Terminator
  ThermDeiceReq_Terminator : Terminator
  ThermProtnSts_Terminator : Terminator
  ThermRfgModReq_Terminator : Terminator
  ThermRfgModSts_Terminator : Terminator
  ThermRfgModSwtSts_Terminator : Terminator
  ThermSysSts_Terminator : Terminator
  UsgModSts_Terminator : Terminator
  VehMktForPmSnsrAirMtrlSnsrReq_Terminator : Terminator
  VehMktForPmSnsrVehMktGlb_Terminator : Terminator
  VehSpd_Terminator : Terminator
  VentReq_FL_Terminator : Terminator
  VentReq_FR_Terminator : Terminator
  VentReq_RL_Terminator : Terminator
  WhlMotCooltFlowMinReq_Terminator : Terminator
  WhlMotCooltFlwEstimd_Terminator : Terminator
  WhlMotSysCoolgReq_Terminator : Terminator
  WhlMotSysCooltT_Terminator : Terminator
  WhlMotSysInvrT_Terminator : Terminator
  WhlMotSysMotT_Terminator : Terminator
  WindLvl_FL_Terminator : Terminator
  WindLvl_FR_Terminator : Terminator
  WindLvl_RL_Terminator : Terminator
  HMI_HMISts_Fr : Outport  OutDataTypeStr=uint8
  HMI_HMISts_Rr : Outport  Port=2  OutDataTypeStr=uint8
  HMI_HMIOnSts_Fr : Outport  Port=3  OutDataTypeStr=uint8
  HMI_HMIOnSts_Rr : Outport  Port=4  OutDataTypeStr=uint8
  HMI_OnOffDsp_Fr : Outport  Port=5  OutDataTypeStr=uint8
  HMI_OnOffDsp_Rr : Outport  Port=6  OutDataTypeStr=uint8
  HMI_AutoManuDsp_Fr : Outport  Port=7  OutDataTypeStr=uint8
  HMI_AutoManuDsp_Rr : Outport  Port=8  OutDataTypeStr=uint8
  HMI_MaxDefDsp : Outport  Port=9  OutDataTypeStr=uint8
  HMI_MaxACDsp_Fr : Outport  Port=10  OutDataTypeStr=uint8
  HMI_MaxHeatDsp_Fr : Outport  Port=11  OutDataTypeStr=uint8
  HMI_FastVentDsp : Outport  Port=12  OutDataTypeStr=uint8
  HMI_MaxACDsp_Rr : Outport  Port=13  OutDataTypeStr=uint8
  HMI_MaxHeatDsp_Rr : Outport  Port=14  OutDataTypeStr=uint8
  HMI_AC_Fr : Outport  Port=15  OutDataTypeStr=uint8
  HMI_AC_Rr : Outport  Port=16  OutDataTypeStr=uint8
  HMI_ACDsp_Fr : Outport  Port=17  OutDataTypeStr=uint8
  HMI_ACDsp_Rr : Outport  Port=18  OutDataTypeStr=uint8
  HMI_Heat_Fr : Outport  Port=19  OutDataTypeStr=uint8
  HMI_Heat_Rr : Outport  Port=20  OutDataTypeStr=uint8
  HMI_HeatDsp_Fr : Outport  Port=21  OutDataTypeStr=uint8
  HMI_HeatDsp_Rr : Outport  Port=22  OutDataTypeStr=uint8
  HMI_Vent_Fr : Outport  Port=23  OutDataTypeStr=uint8
  HMI_Vent_Rr : Outport  Port=24  OutDataTypeStr=uint8
  HMI_VentDsp_Fr : Outport  Port=25  OutDataTypeStr=uint8
  HMI_VentDsp_Rr : Outport  Port=26  OutDataTypeStr=uint8
  HMI_TSet_FL : Outport  Port=27  OutDataTypeStr=uint16
  HMI_TSet_FR : Outport  Port=28  OutDataTypeStr=uint16
  HMI_TSet_Rr : Outport  Port=29  OutDataTypeStr=uint16
  HMI_TSetDsp_FL : Outport  Port=30  OutDataTypeStr=uint16
  HMI_TSetDsp_FR : Outport  Port=31  OutDataTypeStr=uint16
  HMI_TSetDsp_Rr : Outport  Port=32  OutDataTypeStr=uint16
  HMI_WindLvl_FL : Outport  Port=33  OutDataTypeStr=uint8
  HMI_WindLvl_FR : Outport  Port=34  OutDataTypeStr=uint8
  HMI_WindLvl_Rr : Outport  Port=35  OutDataTypeStr=uint8
  HMI_WindLvlDsp_FL : Outport  Port=36  OutDataTypeStr=uint8
  HMI_WindLvlDsp_FR : Outport  Port=37  OutDataTypeStr=uint8
  HMI_WindLvlDsp_Rr : Outport  Port=38  OutDataTypeStr=uint8
  HMI_OutletMode_Fr : Outport  Port=39  OutDataTypeStr=uint8
  HMI_OutletMode_Rr : Outport  Port=40  OutDataTypeStr=uint8
  HMI_OutletModeDsp_Fr : Outport  Port=41  OutDataTypeStr=uint8
  HMI_OutletModeDsp_Rr : Outport  Port=42  OutDataTypeStr=uint8
  HMI_Sync : Outport  Port=43  OutDataTypeStr=uint8
  HMI_SyncDsp : Outport  Port=44  OutDataTypeStr=uint8
  HMI_Inlet : Outport  Port=45  OutDataTypeStr=uint8
  HMI_InletDsp : Outport  Port=46  OutDataTypeStr=uint8
  HMI_ECO : Outport  Port=47  OutDataTypeStr=uint8
  HMI_ECODsp : Outport  Port=48  OutDataTypeStr=uint8
  HMI_AQS : Outport  Port=49  OutDataTypeStr=uint8
  HMI_AQSDsp : Outport  Port=50  OutDataTypeStr=uint8
  HMI_RrWndHet : Outport  Port=51  OutDataTypeStr=uint8
  HMI_RrWndHetDsp : Outport  Port=52  OutDataTypeStr=uint8
  HMI_CfgAutoWindLvl : Outport  Port=53  OutDataTypeStr=uint8
  HMI_CfgAutoWindLvlDsp : Outport  Port=54  OutDataTypeStr=uint8
  HMI_ACFrtPnlLckRrPnlDsp : Outport  Port=55  OutDataTypeStr=uint8
  IoTx_FrntBlwPwmCmd_u16 : Outport  Port=56  OutDataTypeStr=uint16
  IoTx_FrntBlwFrqCmd_u16 : Outport  Port=57  OutDataTypeStr=uint16
  IoTx_DCMot1RunDir_u8 : Outport  Port=58  OutDataTypeStr=uint8
  IoTx_DCMot2RunDir_u8 : Outport  Port=59  OutDataTypeStr=uint8
  IoTx_DCMot3RunDir_u8 : Outport  Port=60  OutDataTypeStr=uint8
  IoTx_DCMot4RunDir_u8 : Outport  Port=61  OutDataTypeStr=uint8
  IoTx_DCMot5RunDir_u8 : Outport  Port=62  OutDataTypeStr=uint8
  IoTx_DCMot6RunDir_u8 : Outport  Port=63  OutDataTypeStr=uint8
  IoTx_DCMot7RunDir_u8 : Outport  Port=64  OutDataTypeStr=uint8
  IoTx_DCMot1PwmCmd_u16 : Outport  Port=65  OutDataTypeStr=uint16
  IoTx_DCMot2PwmCmd_u16 : Outport  Port=66  OutDataTypeStr=uint16
  IoTx_DCMot3PwmCmd_u16 : Outport  Port=67  OutDataTypeStr=uint16
  IoTx_DCMot4PwmCmd_u16 : Outport  Port=68  OutDataTypeStr=uint16
  IoTx_DCMot5PwmCmd_u16 : Outport  Port=69  OutDataTypeStr=uint16
  IoTx_DCMot6PwmCmd_u16 : Outport  Port=70  OutDataTypeStr=uint16
  IoTx_DCMot7PwmCmd_u16 : Outport  Port=71  OutDataTypeStr=uint16
  IoTx_DCMot1FrqCmd_u16 : Outport  Port=72  OutDataTypeStr=uint16
  IoTx_DCMot2FrqCmd_u16 : Outport  Port=73  OutDataTypeStr=uint16
  IoTx_DCMot3FrqCmd_u16 : Outport  Port=74  OutDataTypeStr=uint16
  IoTx_DCMot4FrqCmd_u16 : Outport  Port=75  OutDataTypeStr=uint16
  IoTx_DCMot5FrqCmd_u16 : Outport  Port=76  OutDataTypeStr=uint16
  IoTx_DCMot6FrqCmd_u16 : Outport  Port=77  OutDataTypeStr=uint16
  IoTx_DCMot7FrqCmd_u16 : Outport  Port=78  OutDataTypeStr=uint16
  IoTx_FrntCbnTFanRly_b : Outport  Port=79  OutDataTypeStr=boolean
  IoTx_ClimtRly_b : Outport  Port=80  OutDataTypeStr=boolean
  IoTx_ClimtPwrRly_b : Outport  Port=81  OutDataTypeStr=boolean
  IoTx_HvBattPmpPwmCmd_u16 : Outport  Port=82  OutDataTypeStr=uint16
  IoTx_HvBattPmpFrqCmd_u16 : Outport  Port=83  OutDataTypeStr=uint16
  IoTx_EldtPmpPwmCmd_u16 : Outport  Port=84  OutDataTypeStr=uint16
  IoTx_EldtPmpFrqCmd_u16 : Outport  Port=85  OutDataTypeStr=uint16
  IoTx_HeatrPmpPwmCmd_u16 : Outport  Port=86  OutDataTypeStr=uint16
  IoTx_HeatrPmpFrqCmd_u16 : Outport  Port=87  OutDataTypeStr=uint16
  IoTx_CoolgFanPwmCmd_u16 : Outport  Port=88  OutDataTypeStr=uint16
  IoTx_CoolgFanFrqCmd_u16 : Outport  Port=89  OutDataTypeStr=uint16
  IoTx_SOV1Rly_b : Outport  Port=90  OutDataTypeStr=boolean
  IoTx_SOV2Rly_b : Outport  Port=91  OutDataTypeStr=boolean
  IoTx_SOV3Rly_b : Outport  Port=92  OutDataTypeStr=boolean
  IoTx_ThermPwr1Rly_b : Outport  Port=93  OutDataTypeStr=boolean
  IoTx_ThermPwr2Rly_b : Outport  Port=94  OutDataTypeStr=boolean
  IoTx_ThermPwr3Rly_b : Outport  Port=95  OutDataTypeStr=boolean
  IoTx_CoolgFanRly_b : Outport  Port=96  OutDataTypeStr=boolean
  IoTx_PmpRly_b : Outport  Port=97  OutDataTypeStr=boolean
  wires:
  HMI_HMISts_Fr_Ground/1 -> HMI_HMISts_Fr/1
  HMI_HMISts_Rr_Ground/1 -> HMI_HMISts_Rr/1
  HMI_HMIOnSts_Fr_Ground/1 -> HMI_HMIOnSts_Fr/1
  HMI_HMIOnSts_Rr_Ground/1 -> HMI_HMIOnSts_Rr/1
  HMI_OnOffDsp_Fr_Ground/1 -> HMI_OnOffDsp_Fr/1
  HMI_OnOffDsp_Rr_Ground/1 -> HMI_OnOffDsp_Rr/1
  HMI_AutoManuDsp_Fr_Ground/1 -> HMI_AutoManuDsp_Fr/1
  HMI_AutoManuDsp_Rr_Ground/1 -> HMI_AutoManuDsp_Rr/1
  HMI_MaxDefDsp_Ground/1 -> HMI_MaxDefDsp/1
  HMI_MaxACDsp_Fr_Ground/1 -> HMI_MaxACDsp_Fr/1
  HMI_MaxHeatDsp_Fr_Ground/1 -> HMI_MaxHeatDsp_Fr/1
  HMI_FastVentDsp_Ground/1 -> HMI_FastVentDsp/1
  HMI_MaxACDsp_Rr_Ground/1 -> HMI_MaxACDsp_Rr/1
  HMI_MaxHeatDsp_Rr_Ground/1 -> HMI_MaxHeatDsp_Rr/1
  HMI_AC_Fr_Ground/1 -> HMI_AC_Fr/1
  HMI_AC_Rr_Ground/1 -> HMI_AC_Rr/1
  HMI_ACDsp_Fr_Ground/1 -> HMI_ACDsp_Fr/1
  HMI_ACDsp_Rr_Ground/1 -> HMI_ACDsp_Rr/1
  HMI_Heat_Fr_Ground/1 -> HMI_Heat_Fr/1
  HMI_Heat_Rr_Ground/1 -> HMI_Heat_Rr/1
  HMI_HeatDsp_Fr_Ground/1 -> HMI_HeatDsp_Fr/1
  HMI_HeatDsp_Rr_Ground/1 -> HMI_HeatDsp_Rr/1
  HMI_Vent_Fr_Ground/1 -> HMI_Vent_Fr/1
  HMI_Vent_Rr_Ground/1 -> HMI_Vent_Rr/1
  HMI_VentDsp_Fr_Ground/1 -> HMI_VentDsp_Fr/1
  HMI_VentDsp_Rr_Ground/1 -> HMI_VentDsp_Rr/1
  HMI_TSet_FL_Ground/1 -> HMI_TSet_FL/1
  HMI_TSet_FR_Ground/1 -> HMI_TSet_FR/1
  HMI_TSet_Rr_Ground/1 -> HMI_TSet_Rr/1
  HMI_TSetDsp_FL_Ground/1 -> HMI_TSetDsp_FL/1
  HMI_TSetDsp_FR_Ground/1 -> HMI_TSetDsp_FR/1
  HMI_TSetDsp_Rr_Ground/1 -> HMI_TSetDsp_Rr/1
  HMI_WindLvl_FL_Ground/1 -> HMI_WindLvl_FL/1
  HMI_WindLvl_FR_Ground/1 -> HMI_WindLvl_FR/1
  HMI_WindLvl_Rr_Ground/1 -> HMI_WindLvl_Rr/1
  HMI_WindLvlDsp_FL_Ground/1 -> HMI_WindLvlDsp_FL/1
  HMI_WindLvlDsp_FR_Ground/1 -> HMI_WindLvlDsp_FR/1
  HMI_WindLvlDsp_Rr_Ground/1 -> HMI_WindLvlDsp_Rr/1
  HMI_OutletMode_Fr_Ground/1 -> HMI_OutletMode_Fr/1
  HMI_OutletMode_Rr_Ground/1 -> HMI_OutletMode_Rr/1
  HMI_OutletModeDsp_Fr_Ground/1 -> HMI_OutletModeDsp_Fr/1
  HMI_OutletModeDsp_Rr_Ground/1 -> HMI_OutletModeDsp_Rr/1
  HMI_Sync_Ground/1 -> HMI_Sync/1
  HMI_SyncDsp_Ground/1 -> HMI_SyncDsp/1
  HMI_Inlet_Ground/1 -> HMI_Inlet/1
  HMI_InletDsp_Ground/1 -> HMI_InletDsp/1
  HMI_ECO_Ground/1 -> HMI_ECO/1
  HMI_ECODsp_Ground/1 -> HMI_ECODsp/1
  HMI_AQS_Ground/1 -> HMI_AQS/1
  HMI_AQSDsp_Ground/1 -> HMI_AQSDsp/1
  HMI_RrWndHet_Ground/1 -> HMI_RrWndHet/1
  HMI_RrWndHetDsp_Ground/1 -> HMI_RrWndHetDsp/1
  HMI_CfgAutoWindLvl_Ground/1 -> HMI_CfgAutoWindLvl/1
  HMI_CfgAutoWindLvlDsp_Ground/1 -> HMI_CfgAutoWindLvlDsp/1
  HMI_ACFrtPnlLckRrPnlDsp_Ground/1 -> HMI_ACFrtPnlLckRrPnlDsp/1
  OnOffReq_FL/1 -> OnOffReq_FL_Terminator/1
  OnOffReq_FR/1 -> OnOffReq_FR_Terminator/1
  OnOffReq_RL/1 -> OnOffReq_RL_Terminator/1
  AutoReq_FL/1 -> AutoReq_FL_Terminator/1
  AutoReq_FR/1 -> AutoReq_FR_Terminator/1
  AutoReq_RL/1 -> AutoReq_RL_Terminator/1
  MaxDefReq/1 -> MaxDefReq_Terminator/1
  FastVent/1 -> FastVent_Terminator/1
  MaxACReq/1 -> MaxACReq_Terminator/1
  MaxHeatReq/1 -> MaxHeatReq_Terminator/1
  SmartClearReq/1 -> SmartClearReq_Terminator/1
  ACReq_FL/1 -> ACReq_FL_Terminator/1
  ACReq_FR/1 -> ACReq_FR_Terminator/1
  ACReq_RL/1 -> ACReq_RL_Terminator/1
  HeatReq_FL/1 -> HeatReq_FL_Terminator/1
  HeatReq_FR/1 -> HeatReq_FR_Terminator/1
  HeatReq_RL/1 -> HeatReq_RL_Terminator/1
  VentReq_FL/1 -> VentReq_FL_Terminator/1
  VentReq_FR/1 -> VentReq_FR_Terminator/1
  VentReq_RL/1 -> VentReq_RL_Terminator/1
  TSet_FL/1 -> TSet_FL_Terminator/1
  TSet_FR/1 -> TSet_FR_Terminator/1
  TSet_RL/1 -> TSet_RL_Terminator/1
  WindLvl_FL/1 -> WindLvl_FL_Terminator/1
  WindLvl_FR/1 -> WindLvl_FR_Terminator/1
  WindLvl_RL/1 -> WindLvl_RL_Terminator/1
  OutletMode_FL/1 -> OutletMode_FL_Terminator/1
  OutletMode_FR/1 -> OutletMode_FR_Terminator/1
  OutletMode_RL/1 -> OutletMode_RL_Terminator/1
  Sync/1 -> Sync_Terminator/1
  Inlet/1 -> Inlet_Terminator/1
  ECO/1 -> ECO_Terminator/1
  AQS/1 -> AQS_Terminator/1
  RrWndHet/1 -> RrWndHet_Terminator/1
  CfgAutoWindLvl/1 -> CfgAutoWindLvl_Terminator/1
  ACFrtPnlLckRrPnl/1 -> ACFrtPnlLckRrPnl_Terminator/1
  OccupantStsFL/1 -> OccupantStsFL_Terminator/1
  OccupantStsFR/1 -> OccupantStsFR_Terminator/1
  OccupantStsRL/1 -> OccupantStsRL_Terminator/1
  OccupantStsRM/1 -> OccupantStsRM_Terminator/1
  OccupantStsRR/1 -> OccupantStsRR_Terminator/1
  CmptmtFrntWindDewT/1 -> CmptmtFrntWindDewT_Terminator/1
  CmptmtFrntWindT/1 -> CmptmtFrntWindT_Terminator/1
  CmptmtRelHum/1 -> CmptmtRelHum_Terminator/1
  RiSolarData/1 -> RiSolarData_Terminator/1
  LeSolarData/1 -> LeSolarData_Terminator/1
  VehSpd/1 -> VehSpd_Terminator/1
  CarModSts/1 -> CarModSts_Terminator/1
  UsgModSts/1 -> UsgModSts_Terminator/1
  Cal_Sig_AmbTEna/1 -> Cal_Sig_AmbTEna_Terminator/1
  Cal_Sig_AmbT/1 -> Cal_Sig_AmbT_Terminator/1
  Cal_Sig_InCarTEna/1 -> Cal_Sig_InCarTEna_Terminator/1
  Cal_Sig_InCarT/1 -> Cal_Sig_InCarT_Terminator/1
  Cal_Sig_HvacEvaprTFrntEna/1 -> Cal_Sig_HvacEvaprTFrntEna_Terminator/1
  Cal_Sig_HvacEvaprTFrntT/1 -> Cal_Sig_HvacEvaprTFrntT_Terminator/1
  Cal_Sig_HvacEvaprTReEna/1 -> Cal_Sig_HvacEvaprTReEna_Terminator/1
  Cal_Sig_HvacEvaprTReT/1 -> Cal_Sig_HvacEvaprTReT_Terminator/1
  Cal_Sig_HvacCondsorTFrntTEna/1 -> Cal_Sig_HvacCondsorTFrntTEna_Terminator/1
  Cal_Sig_HvacCondsorTFrntT/1 -> Cal_Sig_HvacCondsorTFrntT_Terminator/1
  Cal_Sig_CooltT1Ena/1 -> Cal_Sig_CooltT1Ena_Terminator/1
  Cal_Sig_CooltT1/1 -> Cal_Sig_CooltT1_Terminator/1
  Cal_Sig_CooltT2Ena/1 -> Cal_Sig_CooltT2Ena_Terminator/1
  Cal_Sig_CooltT2/1 -> Cal_Sig_CooltT2_Terminator/1
  Cal_Sig_CooltT3Ena/1 -> Cal_Sig_CooltT3Ena_Terminator/1
  Cal_Sig_CooltT3/1 -> Cal_Sig_CooltT3_Terminator/1
  AutoDeHumPopUp/1 -> AutoDeHumPopUp_Terminator/1
  AutoDefrstPopUp/1 -> AutoDefrstPopUp_Terminator/1
  AutoFreshPopUp/1 -> AutoFreshPopUp_Terminator/1
  ClimaDefrstSts/1 -> ClimaDefrstSts_Terminator/1
  ClimaDefrstMaxSts/1 -> ClimaDefrstMaxSts_Terminator/1
  HvacFrntBlowerSts/1 -> HvacFrntBlowerSts_Terminator/1
  HvacReBlowerSts/1 -> HvacReBlowerSts_Terminator/1
  HvacAirMFlwFrntEstimd/1 -> HvacAirMFlwFrntEstimd_Terminator/1
  HvacAirMFlwReEstimd/1 -> HvacAirMFlwReEstimd_Terminator/1
  HvacAirQFlwFrntEstimd/1 -> HvacAirQFlwFrntEstimd_Terminator/1
  HvacAirQFlwReEstimd/1 -> HvacAirQFlwReEstimd_Terminator/1
  HvacFrntBlwSpdFb/1 -> HvacFrntBlwSpdFb_Terminator/1
  HvacReBlwSpdFb/1 -> HvacReBlwSpdFb_Terminator/1
  HvacCoolgEnaFrnt/1 -> HvacCoolgEnaFrnt_Terminator/1
  HvacCoolgEnaRe/1 -> HvacCoolgEnaRe_Terminator/1
  HvacDefrstFlapActlPosn/1 -> HvacDefrstFlapActlPosn_Terminator/1
  HvacEvaprTSpFrnt/1 -> HvacEvaprTSpFrnt_Terminator/1
  HvacEvaprTSpRe/1 -> HvacEvaprTSpRe_Terminator/1
  HvacModFlapActlPosnFrstRowLe/1 -> HvacModFlapActlPosnFrstRowLe_Terminator/1
  HvacModFlapActlPosnFrstRowRi/1 -> HvacModFlapActlPosnFrstRowRi_Terminator/1
  HvacModFlapActlPosnSecRowLe/1 -> HvacModFlapActlPosnSecRowLe_Terminator/1
  HvacModFlapActlPosnSecRowRi/1 -> HvacModFlapActlPosnSecRowRi_Terminator/1
  HvacOsaFlapActlPosn/1 -> HvacOsaFlapActlPosn_Terminator/1
  HvacRecFlapActlPosn/1 -> HvacRecFlapActlPosn_Terminator/1
  HvacRecircActRat/1 -> HvacRecircActRat_Terminator/1
  HvacTempFlapActlPosnFrstRowLe/1 -> HvacTempFlapActlPosnFrstRowLe_Terminator/1
  HvacTempFlapActlPosnFrstRowRi/1 -> HvacTempFlapActlPosnFrstRowRi_Terminator/1
  HvacTempFlapActlPosnSecRowLe/1 -> HvacTempFlapActlPosnSecRowLe_Terminator/1
  HvacTempFlapActlPosnSecRowRi/1 -> HvacTempFlapActlPosnSecRowRi_Terminator/1
  HvacTgtAirTForRowFirstLe/1 -> HvacTgtAirTForRowFirstLe_Terminator/1
  HvacTgtAirTForRowFirstRi/1 -> HvacTgtAirTForRowFirstRi_Terminator/1
  HvacTgtAirTForRowSecLe/1 -> HvacTgtAirTForRowSecLe_Terminator/1
  HvacTgtAirTForRowSecRi/1 -> HvacTgtAirTForRowSecRi_Terminator/1
  AmbTEstimdAmbTEstimd/1 -> AmbTEstimdAmbTEstimd_Terminator/1
  AmbTEstimdQf/1 -> AmbTEstimdQf_Terminator/1
  CmptmtTFrntCmptmtTFrnt/1 -> CmptmtTFrntCmptmtTFrnt_Terminator/1
  CmptmtTFrntFanForCmptmtTRunng/1 -> CmptmtTFrntFanForCmptmtTRunng_Terminator/1
  CmptmtTFrntQf/1 -> CmptmtTFrntQf_Terminator/1
  CmptmtTReCmptmtTFrnt/1 -> CmptmtTReCmptmtTFrnt_Terminator/1
  CmptmtTReCmptmtTFrntQf/1 -> CmptmtTReCmptmtTFrntQf_Terminator/1
  CmptmtTReFanForCmptmtTRunng/1 -> CmptmtTReFanForCmptmtTRunng_Terminator/1
  HvacEvaprTFrntTHvac/1 -> HvacEvaprTFrntTHvac_Terminator/1
  HvacEvaprTFrntTQf/1 -> HvacEvaprTFrntTQf_Terminator/1
  HvacEvaprTReTHvac/1 -> HvacEvaprTReTHvac_Terminator/1
  HvacEvaprTReTQf/1 -> HvacEvaprTReTQf_Terminator/1
  HvacAirTForRowFirstAtFlrLeTHvac/1 -> HvacAirTForRowFirstAtFlrLeTHvac_Terminator/1
  HvacAirTForRowFirstAtFlrLeTQf/1 -> HvacAirTForRowFirstAtFlrLeTQf_Terminator/1
  HvacAirTForRowFirstAtFlrRiTHvac/1 -> HvacAirTForRowFirstAtFlrRiTHvac_Terminator/1
  HvacAirTForRowFirstAtFlrRiTQf/1 -> HvacAirTForRowFirstAtFlrRiTQf_Terminator/1
  HvacAirTForRowFirstAtFaceLeTHvac/1 -> HvacAirTForRowFirstAtFaceLeTHvac_Terminator/1
  HvacAirTForRowFirstAtFaceLeTQf/1 -> HvacAirTForRowFirstAtFaceLeTQf_Terminator/1
  HvacAirTForRowFirstAtFaceRiTHvac/1 -> HvacAirTForRowFirstAtFaceRiTHvac_Terminator/1
  HvacAirTForRowFirstAtFaceRiTQf/1 -> HvacAirTForRowFirstAtFaceRiTQf_Terminator/1
  HvacAirTForRowSecAtFlrLeTHvac/1 -> HvacAirTForRowSecAtFlrLeTHvac_Terminator/1
  HvacAirTForRowSecAtFlrLeTQf/1 -> HvacAirTForRowSecAtFlrLeTQf_Terminator/1
  HvacAirTForRowSecAtFlrRiTHvac/1 -> HvacAirTForRowSecAtFlrRiTHvac_Terminator/1
  HvacAirTForRowSecAtFlrRiTQf/1 -> HvacAirTForRowSecAtFlrRiTQf_Terminator/1
  HvacAirTForRowSecAtFaceLeTHvac/1 -> HvacAirTForRowSecAtFaceLeTHvac_Terminator/1
  HvacAirTForRowSecAtFaceLeTQf/1 -> HvacAirTForRowSecAtFaceLeTQf_Terminator/1
  HvacAirTForRowSecAtFaceRiTHvac/1 -> HvacAirTForRowSecAtFaceRiTHvac_Terminator/1
  HvacAirTForRowSecAtFaceRiTQf/1 -> HvacAirTForRowSecAtFaceRiTQf_Terminator/1
  HvacCondsorTFrntTHvac/1 -> HvacCondsorTFrntTHvac_Terminator/1
  HvacCondsorTFrntTQf/1 -> HvacCondsorTFrntTQf_Terminator/1
  HvacCondsorTspFrntTHvac/1 -> HvacCondsorTspFrntTHvac_Terminator/1
  ClimaThermReq/1 -> ClimaThermReq_Terminator/1
  ClimaThermSts/1 -> ClimaThermSts_Terminator/1
  HvacAirTHvacIntkT/1 -> HvacAirTHvacIntkT_Terminator/1
  RsvdSigForClima01/1 -> RsvdSigForClima01_Terminator/1
  RsvdSigForClima02/1 -> RsvdSigForClima02_Terminator/1
  RsvdSigForClima03/1 -> RsvdSigForClima03_Terminator/1
  RsvdSigForClima04/1 -> RsvdSigForClima04_Terminator/1
  RsvdSigForClima05/1 -> RsvdSigForClima05_Terminator/1
  RsvdSigForClima06/1 -> RsvdSigForClima06_Terminator/1
  RsvdSigForClima07/1 -> RsvdSigForClima07_Terminator/1
  RsvdSigForClima08/1 -> RsvdSigForClima08_Terminator/1
  RsvdSigForClima09/1 -> RsvdSigForClima09_Terminator/1
  RsvdSigForClima10/1 -> RsvdSigForClima10_Terminator/1
  RsvdSigForClima11/1 -> RsvdSigForClima11_Terminator/1
  RsvdSigForClima12/1 -> RsvdSigForClima12_Terminator/1
  RsvdSigForClima13/1 -> RsvdSigForClima13_Terminator/1
  RsvdSigForClima14/1 -> RsvdSigForClima14_Terminator/1
  RsvdSigForClima15/1 -> RsvdSigForClima15_Terminator/1
  RsvdSigForClima16/1 -> RsvdSigForClima16_Terminator/1
  RsvdSigForClima17/1 -> RsvdSigForClima17_Terminator/1
  RsvdSigForClima18/1 -> RsvdSigForClima18_Terminator/1
  RsvdSigForClima19/1 -> RsvdSigForClima19_Terminator/1
  RsvdSigForClima20/1 -> RsvdSigForClima20_Terminator/1
  RsvdSigForClima21/1 -> RsvdSigForClima21_Terminator/1
  RsvdSigForClima22/1 -> RsvdSigForClima22_Terminator/1
  RsvdSigForClima23/1 -> RsvdSigForClima23_Terminator/1
  HvacDefrstFlapTgtPosn/1 -> HvacDefrstFlapTgtPosn_Terminator/1
  HvacModFlapTgtPosnFrstRowLe/1 -> HvacModFlapTgtPosnFrstRowLe_Terminator/1
  HvacModFlapTgtPosnFrstRowRi/1 -> HvacModFlapTgtPosnFrstRowRi_Terminator/1
  HvacModFlapTgtPosnSecRowLe/1 -> HvacModFlapTgtPosnSecRowLe_Terminator/1
  HvacModFlapTgtPosnSecRowRi/1 -> HvacModFlapTgtPosnSecRowRi_Terminator/1
  HvacOsaFlapTgtPosn/1 -> HvacOsaFlapTgtPosn_Terminator/1
  HvacRecFlapTgtPosn/1 -> HvacRecFlapTgtPosn_Terminator/1
  HvacTempFlapTgtPosnFrstRowLe/1 -> HvacTempFlapTgtPosnFrstRowLe_Terminator/1
  HvacTempFlapTgtPosnFrstRowRi/1 -> HvacTempFlapTgtPosnFrstRowRi_Terminator/1
  HvacTempFlapTgtPosnSecRowLe/1 -> HvacTempFlapTgtPosnSecRowLe_Terminator/1
  HvacTempFlapTgtPosnSecRowRi/1 -> HvacTempFlapTgtPosnSecRowRi_Terminator/1
  HvBattThermRunAway/1 -> HvBattThermRunAway_Terminator/1
  WhlMotCooltFlowMinReq/1 -> WhlMotCooltFlowMinReq_Terminator/1
  WhlMotSysCoolgReq/1 -> WhlMotSysCoolgReq_Terminator/1
  WhlMotSysCooltT/1 -> WhlMotSysCooltT_Terminator/1
  WhlMotSysInvrT/1 -> WhlMotSysInvrT_Terminator/1
  WhlMotSysMotT/1 -> WhlMotSysMotT_Terminator/1
  DCChrgSt/1 -> DCChrgSt_Terminator/1
  DCChrgnHndlSts/1 -> DCChrgnHndlSts_Terminator/1
  ACChrgSt/1 -> ACChrgSt_Terminator/1
  ACChrgnHndlSts/1 -> ACChrgnHndlSts_Terminator/1
  HvBattCooltFlowReq/1 -> HvBattCooltFlowReq_Terminator/1
  HvBattCooltMaxTReq/1 -> HvBattCooltMaxTReq_Terminator/1
  HvBattCooltMinTReq/1 -> HvBattCooltMinTReq_Terminator/1
  HvBattCooltTReq/1 -> HvBattCooltTReq_Terminator/1
  HvBattThermReq/1 -> HvBattThermReq_Terminator/1
  HvBattTAvg/1 -> HvBattTAvg_Terminator/1
  HvBattTMax/1 -> HvBattTMax_Terminator/1
  HvBattTMin/1 -> HvBattTMin_Terminator/1
  HvBattActSOC/1 -> HvBattActSOC_Terminator/1
  HvSysRlyStsChks/1 -> HvSysRlyStsChks_Terminator/1
  HvSysRlyStsCntr/1 -> HvSysRlyStsCntr_Terminator/1
  HvSysRlyStsHvSysRlySts/1 -> HvSysRlyStsHvSysRlySts_Terminator/1
  HvCmprPwrAllwd/1 -> HvCmprPwrAllwd_Terminator/1
  HvHeatrPwrAllwd/1 -> HvHeatrPwrAllwd_Terminator/1
  WhlMotCooltFlwEstimd/1 -> WhlMotCooltFlwEstimd_Terminator/1
  HvBattCooltFlwEstimd/1 -> HvBattCooltFlwEstimd_Terminator/1
  HvBattThermReqFb/1 -> HvBattThermReqFb_Terminator/1
  HvCmprNormPwrDes/1 -> HvCmprNormPwrDes_Terminator/1
  HvHeatrNormPwrDes/1 -> HvHeatrNormPwrDes_Terminator/1
  HvCmprCritPwrDes/1 -> HvCmprCritPwrDes_Terminator/1
  HvHeatrCritPwrDes/1 -> HvHeatrCritPwrDes_Terminator/1
  ThermDeiceReq/1 -> ThermDeiceReq_Terminator/1
  ThermRfgModReq/1 -> ThermRfgModReq_Terminator/1
  ThermRfgModSts/1 -> ThermRfgModSts_Terminator/1
  ThermRfgModSwtSts/1 -> ThermRfgModSwtSts_Terminator/1
  ThermCooltModReq/1 -> ThermCooltModReq_Terminator/1
  ThermCooltModSts/1 -> ThermCooltModSts_Terminator/1
  ThermCooltModSwtSts/1 -> ThermCooltModSwtSts_Terminator/1
  RfgSnsrT1/1 -> RfgSnsrT1_Terminator/1
  RfgSnsrT2/1 -> RfgSnsrT2_Terminator/1
  RfgSnsrT3/1 -> RfgSnsrT3_Terminator/1
  RfgSnsrT4/1 -> RfgSnsrT4_Terminator/1
  RfgSnsrP1/1 -> RfgSnsrP1_Terminator/1
  RfgSnsrPT1T/1 -> RfgSnsrPT1T_Terminator/1
  RfgSnsrPT1P/1 -> RfgSnsrPT1P_Terminator/1
  RfgSnsrT5Rsvd/1 -> RfgSnsrT5Rsvd_Terminator/1
  RfgSnsrT6Rsvd/1 -> RfgSnsrT6Rsvd_Terminator/1
  RfgSnsrT7Rsvd/1 -> RfgSnsrT7Rsvd_Terminator/1
  RfgSnsrT8Rsvd/1 -> RfgSnsrT8Rsvd_Terminator/1
  RfgSnsrP5Rsvd/1 -> RfgSnsrP5Rsvd_Terminator/1
  RfgSnsrP6Rsvd/1 -> RfgSnsrP6Rsvd_Terminator/1
  RfgSnsrP7Rsvd/1 -> RfgSnsrP7Rsvd_Terminator/1
  RfgSnsrP8Rsvd/1 -> RfgSnsrP8Rsvd_Terminator/1
  CooltSnsrT1/1 -> CooltSnsrT1_Terminator/1
  CooltSnsrT2/1 -> CooltSnsrT2_Terminator/1
  CooltSnsrT3/1 -> CooltSnsrT3_Terminator/1
  CooltSnsrT4Rsvd/1 -> CooltSnsrT4Rsvd_Terminator/1
  CooltSnsrT5Rsvd/1 -> CooltSnsrT5Rsvd_Terminator/1
  CooltSnsrT6Rsvd/1 -> CooltSnsrT6Rsvd_Terminator/1
  CooltSnsrT7Rsvd/1 -> CooltSnsrT7Rsvd_Terminator/1
  CooltSnsrT8Rsvd/1 -> CooltSnsrT8Rsvd_Terminator/1
  CRFMAirMFlwEstimd/1 -> CRFMAirMFlwEstimd_Terminator/1
  CRFMAirQFlwEstimd/1 -> CRFMAirQFlwEstimd_Terminator/1
  ThermCptsSts/1 -> ThermCptsSts_Terminator/1
  ThermProtnSts/1 -> ThermProtnSts_Terminator/1
  ThermSysSts/1 -> ThermSysSts_Terminator/1
  RsvdSigForTherm01/1 -> RsvdSigForTherm01_Terminator/1
  RsvdSigForTherm02/1 -> RsvdSigForTherm02_Terminator/1
  RsvdSigForTherm03/1 -> RsvdSigForTherm03_Terminator/1
  RsvdSigForTherm04/1 -> RsvdSigForTherm04_Terminator/1
  RsvdSigForTherm05/1 -> RsvdSigForTherm05_Terminator/1
  RsvdSigForTherm06/1 -> RsvdSigForTherm06_Terminator/1
  RsvdSigForTherm07/1 -> RsvdSigForTherm07_Terminator/1
  RsvdSigForTherm08/1 -> RsvdSigForTherm08_Terminator/1
  RsvdSigForTherm09/1 -> RsvdSigForTherm09_Terminator/1
  RsvdSigForTherm10/1 -> RsvdSigForTherm10_Terminator/1
  RsvdSigForTherm11/1 -> RsvdSigForTherm11_Terminator/1
  RsvdSigForTherm12/1 -> RsvdSigForTherm12_Terminator/1
  RsvdSigForTherm13/1 -> RsvdSigForTherm13_Terminator/1
  RsvdSigForTherm14/1 -> RsvdSigForTherm14_Terminator/1
  RsvdSigForTherm15/1 -> RsvdSigForTherm15_Terminator/1
  RsvdSigForTherm16/1 -> RsvdSigForTherm16_Terminator/1
  RsvdSigForTherm17/1 -> RsvdSigForTherm17_Terminator/1
  RsvdSigForTherm18/1 -> RsvdSigForTherm18_Terminator/1
  RsvdSigForTherm19/1 -> RsvdSigForTherm19_Terminator/1
  RsvdSigForTherm20/1 -> RsvdSigForTherm20_Terminator/1
  RsvdSigForTherm21/1 -> RsvdSigForTherm21_Terminator/1
  RsvdSigForTherm22/1 -> RsvdSigForTherm22_Terminator/1
  RsvdSigForTherm23/1 -> RsvdSigForTherm23_Terminator/1
  HeatrPmpPwmCmd/1 -> HeatrPmpPwmCmd_Terminator/1
  HvBattPmpPwmCmd/1 -> HvBattPmpPwmCmd_Terminator/1
  EldtPmpPwmCmd/1 -> EldtPmpPwmCmd_Terminator/1
  SOV1OnOffCmd/1 -> SOV1OnOffCmd_Terminator/1
  SOV2OnOffCmd/1 -> SOV2OnOffCmd_Terminator/1
  SOV3OnOffCmd/1 -> SOV3OnOffCmd_Terminator/1
  CoolgFanPWMCmd/1 -> CoolgFanPWMCmd_Terminator/1
  FrntBlwPWMCmd/1 -> FrntBlwPWMCmd_Terminator/1
  BcfvNVMFlt/1 -> BcfvNVMFlt_Terminator/1
  BctvNVMFlt/1 -> BctvNVMFlt_Terminator/1
  CmprEEPROMFault/1 -> CmprEEPROMFault_Terminator/1
  CmprHVoltResonanceStat/1 -> CmprHVoltResonanceStat_Terminator/1
  CmprInCurrOverCurrStat/1 -> CmprInCurrOverCurrStat_Terminator/1
  CmprLiquidSluggingStat/1 -> CmprLiquidSluggingStat_Terminator/1
  CmprLostCommStat/1 -> CmprLostCommStat_Terminator/1
  CmprMotorCurrOverCurrStat/1 -> CmprMotorCurrOverCurrStat_Terminator/1
  CmprOverMotorCurrStat/1 -> CmprOverMotorCurrStat_Terminator/1
  CmprOverPowerStat/1 -> CmprOverPowerStat_Terminator/1
  CmprRAMFault/1 -> CmprRAMFault_Terminator/1
  CmprROMFault/1 -> CmprROMFault_Terminator/1
  CmprReqCmprPwrLim/1 -> CmprReqCmprPwrLim_Terminator/1
  CmprReqCmprRunReq/1 -> CmprReqCmprRunReq_Terminator/1
  CmprReqCmprSpdReq/1 -> CmprReqCmprSpdReq_Terminator/1
  CmprRotorLockStat/1 -> CmprRotorLockStat_Terminator/1
  CmprSpdIncrReq/1 -> CmprSpdIncrReq_Terminator/1
  CooltFlowInCmptmtCirc/1 -> CooltFlowInCmptmtCirc_Terminator/1
  HpBattFwvActvSaveReq/1 -> HpBattFwvActvSaveReq_Terminator/1
  HpBattFwvFltSts/1 -> HpBattFwvFltSts_Terminator/1
  HpBattFwvMode/1 -> HpBattFwvMode_Terminator/1
  HpBattFwvPosRec/1 -> HpBattFwvPosRec_Terminator/1
  HpBattFwvPosSetReq/1 -> HpBattFwvPosSetReq_Terminator/1
  HpBattFwvRefDrvReq/1 -> HpBattFwvRefDrvReq_Terminator/1
  HpBattFwvRunSts/1 -> HpBattFwvRunSts_Terminator/1
  HpBattFwvSpdLvl/1 -> HpBattFwvSpdLvl_Terminator/1
  HpBattFwvSpdLvlReq/1 -> HpBattFwvSpdLvlReq_Terminator/1
  HpBattFwvTempSts/1 -> HpBattFwvTempSts_Terminator/1
  HpBattFwvVoltSts/1 -> HpBattFwvVoltSts_Terminator/1
  HpBattVlvActvSaveReq/1 -> HpBattVlvActvSaveReq_Terminator/1
  HpBattVlvFltSts/1 -> HpBattVlvFltSts_Terminator/1
  HpBattVlvMode/1 -> HpBattVlvMode_Terminator/1
  HpBattVlvPosRec/1 -> HpBattVlvPosRec_Terminator/1
  HpBattVlvPosSetReq/1 -> HpBattVlvPosSetReq_Terminator/1
  HpBattVlvRefDrvReq/1 -> HpBattVlvRefDrvReq_Terminator/1
  HpBattVlvRunSts/1 -> HpBattVlvRunSts_Terminator/1
  HpBattVlvSpdLvl/1 -> HpBattVlvSpdLvl_Terminator/1
  HpBattVlvSpdLvlReq/1 -> HpBattVlvSpdLvlReq_Terminator/1
  HpBattVlvTempSts/1 -> HpBattVlvTempSts_Terminator/1
  HpBattVlvVoltSts/1 -> HpBattVlvVoltSts_Terminator/1
  HvCooltHeatrEnad/1 -> HvCooltHeatrEnad_Terminator/1
  HvCooltHeatrICnsSig/1 -> HvCooltHeatrICnsSig_Terminator/1
  HvCooltHeatrInfoCompProtn/1 -> HvCooltHeatrInfoCompProtn_Terminator/1
  HvCooltHeatrSplyUForCtrlUnitValSig/1 -> HvCooltHeatrSplyUForCtrlUnitValSig_Terminator/1
  HvCooltHeatrStsSig/1 -> HvCooltHeatrStsSig_Terminator/1
  HvCooltWtrHeatrWtrTInIntk/1 -> HvCooltWtrHeatrWtrTInIntk_Terminator/1
  HvCooltWtrHeatrWtrTInOutl/1 -> HvCooltWtrHeatrWtrTInOutl_Terminator/1
  HvHeatrPwrCns/1 -> HvHeatrPwrCns_Terminator/1
  HvHeatrPwrCnsDes/1 -> HvHeatrPwrCnsDes_Terminator/1
  HvWtrHeatrPwrCnsAllwd/1 -> HvWtrHeatrPwrCnsAllwd_Terminator/1
  HvWtrHeatrWtrTDes/1 -> HvWtrHeatrWtrTDes_Terminator/1
  CmprDiagcFbCmprCmprSpdErr/1 -> CmprDiagcFbCmprCmprSpdErr_Terminator/1
  CmprDiagcFbCmprCtrlrErr/1 -> CmprDiagcFbCmprCtrlrErr_Terminator/1
  CmprDiagcFbCmprDrvrCircSnsr/1 -> CmprDiagcFbCmprDrvrCircSnsr_Terminator/1
  CmprDiagcFbCmprDrvrCircSnsrPlaus/1 -> CmprDiagcFbCmprDrvrCircSnsrPlaus_Terminator/1
  CmprDiagcFbCmprHvSnsr1/1 -> CmprDiagcFbCmprHvSnsr1_Terminator/1
  CmprDiagcFbCmprHvSnsr2/1 -> CmprDiagcFbCmprHvSnsr2_Terminator/1
  CmprDiagcFbCmprHvSnsrI/1 -> CmprDiagcFbCmprHvSnsrI_Terminator/1
  CmprDiagcFbCmprHvSnsrICrct/1 -> CmprDiagcFbCmprHvSnsrICrct_Terminator/1
  CmprDiagcFbCmprHvSnsrIPlaus/1 -> CmprDiagcFbCmprHvSnsrIPlaus_Terminator/1
  CmprDiagcFbCmprHvSnsrPlaus/1 -> CmprDiagcFbCmprHvSnsrPlaus_Terminator/1
  CmprDiagcFbCmprHvSplyErr/1 -> CmprDiagcFbCmprHvSplyErr_Terminator/1
  CmprDiagcFbCmprPhaseWire/1 -> CmprDiagcFbCmprPhaseWire_Terminator/1
  CmprDiagcFbCmprT1/1 -> CmprDiagcFbCmprT1_Terminator/1
  CmprDiagcFbCmprT2/1 -> CmprDiagcFbCmprT2_Terminator/1
  CmprDiagcFbCmprTOperErr1/1 -> CmprDiagcFbCmprTOperErr1_Terminator/1
  CmprDiagcFbCmprTOperErr2/1 -> CmprDiagcFbCmprTOperErr2_Terminator/1
  CmprDiagcFbCmprTPlaus/1 -> CmprDiagcFbCmprTPlaus_Terminator/1
  CmprDiagcFbCmprUSplyErr/1 -> CmprDiagcFbCmprUSplyErr_Terminator/1
  CmprFbCmprI/1 -> CmprFbCmprI_Terminator/1
  CmprFbCmprIPha/1 -> CmprFbCmprIPha_Terminator/1
  CmprFbCmprSpd/1 -> CmprFbCmprSpd_Terminator/1
  CmprFbCmprSts1/1 -> CmprFbCmprSts1_Terminator/1
  CmprFbCmprSts2/1 -> CmprFbCmprSts2_Terminator/1
  CmprFbCmprT1/1 -> CmprFbCmprT1_Terminator/1
  CmprFbCmprT2/1 -> CmprFbCmprT2_Terminator/1
  CmprFbCmprU/1 -> CmprFbCmprU_Terminator/1
  EctvCmdVlvMovEna/1 -> EctvCmdVlvMovEna_Terminator/1
  EctvCmdVlvPosSetReq/1 -> EctvCmdVlvPosSetReq_Terminator/1
  EctvCmdVlvSpdLvlReq/1 -> EctvCmdVlvSpdLvlReq_Terminator/1
  EctvStatVlvFaultSts/1 -> EctvStatVlvFaultSts_Terminator/1
  EctvStatVlvPosSts/1 -> EctvStatVlvPosSts_Terminator/1
  EctvStatVlvRunSts/1 -> EctvStatVlvRunSts_Terminator/1
  EctvStatVlvSpdLvl/1 -> EctvStatVlvSpdLvl_Terminator/1
  EctvStatVlvTempSts/1 -> EctvStatVlvTempSts_Terminator/1
  EctvStatVoltSts/1 -> EctvStatVoltSts_Terminator/1
  HvCooltHeatrEnadWhE2EChks/1 -> HvCooltHeatrEnadWhE2EChks_Terminator/1
  HvCooltHeatrEnadWhE2ECntr/1 -> HvCooltHeatrEnadWhE2ECntr_Terminator/1
  HvCooltHeatrEnadWhE2EHvchEnad/1 -> HvCooltHeatrEnadWhE2EHvchEnad_Terminator/1
  HvCooltHeatrProtnOfSelfTmpSigHwProtn/1 -> HvCooltHeatrProtnOfSelfTmpSigHwProtn_Terminator/1
  HvCooltHeatrProtnOfSelfTmpSigOvrheatg/1 -> HvCooltHeatrProtnOfSelfTmpSigOvrheatg_Terminator/1
  HvCooltHeatrProtnOfSelfTmpSigProtnOfSelfTmp/1 -> HvCooltHeatrProtnOfSelfTmpSigProtnOfSelfTmp_Terminator/1
  HvCooltHeatrProtnOfSelfTmpSigProtnOfSelfTmpResd/1 -> HvCooltHeatrProtnOfSelfTmpSigProtnOfSelfTmpResd_Terminator/1
  HvCooltHeatrSnsrFltSigCooltTInSnsrFlt/1 -> HvCooltHeatrSnsrFltSigCooltTInSnsrFlt_Terminator/1
  HvCooltHeatrSnsrFltSigCooltTOutSnsrFlt/1 -> HvCooltHeatrSnsrFltSigCooltTOutSnsrFlt_Terminator/1
  HvCooltHeatrSnsrFltSigResdForSnsrFlt/1 -> HvCooltHeatrSnsrFltSigResdForSnsrFlt_Terminator/1
  HvCooltHeatrSnsrFltSigTInMtrlSnsrFlt/1 -> HvCooltHeatrSnsrFltSigTInMtrlSnsrFlt_Terminator/1
  HvCooltHeatrSrvRqrdSigCircForDrvrShoOrOpen/1 -> HvCooltHeatrSrvRqrdSigCircForDrvrShoOrOpen_Terminator/1
  HvCooltHeatrSrvRqrdSigICnsOutOfRng/1 -> HvCooltHeatrSrvRqrdSigICnsOutOfRng_Terminator/1
  HvCooltHeatrSrvRqrdSigMemErr/1 -> HvCooltHeatrSrvRqrdSigMemErr_Terminator/1
  HvCooltHeatrSrvRqrdSigSrvRqrd/1 -> HvCooltHeatrSrvRqrdSigSrvRqrd_Terminator/1
  HvCooltHeatrSrvRqrdSigSrvRqrdResd/1 -> HvCooltHeatrSrvRqrdSigSrvRqrdResd_Terminator/1
  HvCooltHeatrStsWhE2EChks/1 -> HvCooltHeatrStsWhE2EChks_Terminator/1
  HvCooltHeatrStsWhE2ECntr/1 -> HvCooltHeatrStsWhE2ECntr_Terminator/1
  HvCooltHeatrStsWhE2EHvchSts/1 -> HvCooltHeatrStsWhE2EHvchSts_Terminator/1
  HvCooltHeatrWarnSigCooltTOutOfRng/1 -> HvCooltHeatrWarnSigCooltTOutOfRng_Terminator/1
  HvCooltHeatrWarnSigFltInCom/1 -> HvCooltHeatrWarnSigFltInCom_Terminator/1
  HvCooltHeatrWarnSigFltPrsnt/1 -> HvCooltHeatrWarnSigFltPrsnt_Terminator/1
  HvCooltHeatrWarnSigFltPrsntResd/1 -> HvCooltHeatrWarnSigFltPrsntResd_Terminator/1
  HvCooltHeatrWarnSigHvOutOfRng/1 -> HvCooltHeatrWarnSigHvOutOfRng_Terminator/1
  HvCooltHeatrWarnSigULoOutOfRng/1 -> HvCooltHeatrWarnSigULoOutOfRng_Terminator/1
  BexvNVMFlt/1 -> BexvNVMFlt_Terminator/1
  CexvNVMFlt/1 -> CexvNVMFlt_Terminator/1
  EexvNVMFlt/1 -> EexvNVMFlt_Terminator/1
  BexvPosnReqExvCalibReq/1 -> BexvPosnReqExvCalibReq_Terminator/1
  BexvPosnReqExvHeatdReq/1 -> BexvPosnReqExvHeatdReq_Terminator/1
  BexvPosnReqExvMovEnable/1 -> BexvPosnReqExvMovEnable_Terminator/1
  BexvPosnReqExvPosnReq/1 -> BexvPosnReqExvPosnReq_Terminator/1
  BexvStsExvActrPosn/1 -> BexvStsExvActrPosn_Terminator/1
  BexvStsExvBlkErr/1 -> BexvStsExvBlkErr_Terminator/1
  BexvStsExvCalibSts/1 -> BexvStsExvCalibSts_Terminator/1
  BexvStsExvElecStsErr/1 -> BexvStsExvElecStsErr_Terminator/1
  BexvStsExvMovSts/1 -> BexvStsExvMovSts_Terminator/1
  BexvStsExvOvrTempErr/1 -> BexvStsExvOvrTempErr_Terminator/1
  BexvStsExvOvrTrvlErr/1 -> BexvStsExvOvrTrvlErr_Terminator/1
  BexvStsExvPreHeatgSts/1 -> BexvStsExvPreHeatgSts_Terminator/1
  BexvStsExvVoltgRangErr/1 -> BexvStsExvVoltgRangErr_Terminator/1
  CexvPosnReqExvCalibReq/1 -> CexvPosnReqExvCalibReq_Terminator/1
  CexvPosnReqExvHeatdReq/1 -> CexvPosnReqExvHeatdReq_Terminator/1
  CexvPosnReqExvMovEnable/1 -> CexvPosnReqExvMovEnable_Terminator/1
  CexvPosnReqExvPosnReq/1 -> CexvPosnReqExvPosnReq_Terminator/1
  CexvStsExvActrPosn/1 -> CexvStsExvActrPosn_Terminator/1
  CexvStsExvBlkErr/1 -> CexvStsExvBlkErr_Terminator/1
  CexvStsExvCalibSts/1 -> CexvStsExvCalibSts_Terminator/1
  CexvStsExvElecStsErr/1 -> CexvStsExvElecStsErr_Terminator/1
  CexvStsExvMovSts/1 -> CexvStsExvMovSts_Terminator/1
  CexvStsExvOvrTempErr/1 -> CexvStsExvOvrTempErr_Terminator/1
  CexvStsExvOvrTrvlErr/1 -> CexvStsExvOvrTrvlErr_Terminator/1
  CexvStsExvPreHeatgSts/1 -> CexvStsExvPreHeatgSts_Terminator/1
  CexvStsExvVoltgRangErr/1 -> CexvStsExvVoltgRangErr_Terminator/1
  EexvPosnReqExvCalibReq/1 -> EexvPosnReqExvCalibReq_Terminator/1
  EexvPosnReqExvHeatdReq/1 -> EexvPosnReqExvHeatdReq_Terminator/1
  EexvPosnReqExvMovEnable/1 -> EexvPosnReqExvMovEnable_Terminator/1
  EexvPosnReqExvPosnReq/1 -> EexvPosnReqExvPosnReq_Terminator/1
  EexvStsExvActrPosn/1 -> EexvStsExvActrPosn_Terminator/1
  EexvStsExvBlkErr/1 -> EexvStsExvBlkErr_Terminator/1
  EexvStsExvCalibSts/1 -> EexvStsExvCalibSts_Terminator/1
  EexvStsExvElecStsErr/1 -> EexvStsExvElecStsErr_Terminator/1
  EexvStsExvMovSts/1 -> EexvStsExvMovSts_Terminator/1
  EexvStsExvOvrTempErr/1 -> EexvStsExvOvrTempErr_Terminator/1
  EexvStsExvOvrTrvlErr/1 -> EexvStsExvOvrTrvlErr_Terminator/1
  EexvStsExvPreHeatgSts/1 -> EexvStsExvPreHeatgSts_Terminator/1
  EexvStsExvVoltgRangErr/1 -> EexvStsExvVoltgRangErr_Terminator/1
  AGMNVMFlt/1 -> AGMNVMFlt_Terminator/1
  GrlActTrqBoost/1 -> GrlActTrqBoost_Terminator/1
  GrlAutoCalibReq/1 -> GrlAutoCalibReq_Terminator/1
  GrlHldTrqActive/1 -> GrlHldTrqActive_Terminator/1
  GrlShttrMoveActive/1 -> GrlShttrMoveActive_Terminator/1
  GrlShttrOverVolt/1 -> GrlShttrOverVolt_Terminator/1
  GrlShttrOvertravelErr/1 -> GrlShttrOvertravelErr_Terminator/1
  GrlTrqBoostReq/1 -> GrlTrqBoostReq_Terminator/1
  GrlShttrDmdShttrCalEna/1 -> GrlShttrDmdShttrCalEna_Terminator/1
  GrlShttrDmdShttrPosnReq/1 -> GrlShttrDmdShttrPosnReq_Terminator/1
  GrlShttrStsShttrActrFlt/1 -> GrlShttrStsShttrActrFlt_Terminator/1
  GrlShttrStsShttrBlkd/1 -> GrlShttrStsShttrBlkd_Terminator/1
  GrlShttrStsShttrCalActv/1 -> GrlShttrStsShttrCalActv_Terminator/1
  GrlShttrStsShttrCalIndcd/1 -> GrlShttrStsShttrCalIndcd_Terminator/1
  GrlShttrStsShttrElecErr/1 -> GrlShttrStsShttrElecErr_Terminator/1
  GrlShttrStsShttrPosnRaw/1 -> GrlShttrStsShttrPosnRaw_Terminator/1
  GrlShttrStsShttrSnsrFlt/1 -> GrlShttrStsShttrSnsrFlt_Terminator/1
  GrlShttrStsShttrTErr/1 -> GrlShttrStsShttrTErr_Terminator/1
  GrlShttrStsShttrULoErr/1 -> GrlShttrStsShttrULoErr_Terminator/1
  AFUGenErr/1 -> AFUGenErr_Terminator/1
  AirFragActEnad/1 -> AirFragActEnad_Terminator/1
  AirFragCh1/1 -> AirFragCh1_Terminator/1
  AirFragCh1AvlTi/1 -> AirFragCh1AvlTi_Terminator/1
  AirFragCh1RunngSts/1 -> AirFragCh1RunngSts_Terminator/1
  AirFragCh1Type/1 -> AirFragCh1Type_Terminator/1
  AirFragCh2/1 -> AirFragCh2_Terminator/1
  AirFragCh2AvlTi/1 -> AirFragCh2AvlTi_Terminator/1
  AirFragCh2RunngSts/1 -> AirFragCh2RunngSts_Terminator/1
  AirFragCh2Type/1 -> AirFragCh2Type_Terminator/1
  AirFragCh3/1 -> AirFragCh3_Terminator/1
  AirFragCh3AvlTi/1 -> AirFragCh3AvlTi_Terminator/1
  AirFragCh3RunngSts/1 -> AirFragCh3RunngSts_Terminator/1
  AirFragCh3Type/1 -> AirFragCh3Type_Terminator/1
  AirFragCh4/1 -> AirFragCh4_Terminator/1
  AirFragCh4AvlTi/1 -> AirFragCh4AvlTi_Terminator/1
  AirFragCh4RunngSts/1 -> AirFragCh4RunngSts_Terminator/1
  AirFragCh4Type/1 -> AirFragCh4Type_Terminator/1
  AirFragCh5/1 -> AirFragCh5_Terminator/1
  AirFragCh5AvlTi/1 -> AirFragCh5AvlTi_Terminator/1
  AirFragCh5RunngSts/1 -> AirFragCh5RunngSts_Terminator/1
  AirFragCh5Type/1 -> AirFragCh5Type_Terminator/1
  AirFragChgSts/1 -> AirFragChgSts_Terminator/1
  AirFragConcReq/1 -> AirFragConcReq_Terminator/1
  AirFragFanErr/1 -> AirFragFanErr_Terminator/1
  AirFragInitSts/1 -> AirFragInitSts_Terminator/1
  AirFragLvlRspn/1 -> AirFragLvlRspn_Terminator/1
  AirFragMot1Err/1 -> AirFragMot1Err_Terminator/1
  AirFragMot2Err/1 -> AirFragMot2Err_Terminator/1
  AirFragMot3Err/1 -> AirFragMot3Err_Terminator/1
  AirFragMot4Err/1 -> AirFragMot4Err_Terminator/1
  AirFragMot5Err/1 -> AirFragMot5Err_Terminator/1
  AirFragOvrVoltErr/1 -> AirFragOvrVoltErr_Terminator/1
  AirFragTempErr/1 -> AirFragTempErr_Terminator/1
  AirFragUndVoltErr/1 -> AirFragUndVoltErr_Terminator/1
  CmpmtInAirPmAQI/1 -> CmpmtInAirPmAQI_Terminator/1
  CmpmtInAirPmDnsty/1 -> CmpmtInAirPmDnsty_Terminator/1
  HvacAirMFlowVent/1 -> HvacAirMFlowVent_Terminator/1
  HvacRecircAct/1 -> HvacRecircAct_Terminator/1
  InPm25FanErr/1 -> InPm25FanErr_Terminator/1
  InPm25SensrIntErr/1 -> InPm25SensrIntErr_Terminator/1
  InPm25SnrTempErr/1 -> InPm25SnrTempErr_Terminator/1
  InPm25SnrVoltgRangErr/1 -> InPm25SnrVoltgRangErr_Terminator/1
  InPm25SnsrActnReq/1 -> InPm25SnsrActnReq_Terminator/1
  InPm25SnsrElecErr/1 -> InPm25SnsrElecErr_Terminator/1
  InPm25SnsrSts/1 -> InPm25SnsrSts_Terminator/1
  CmptmtAirTEstimdExtdComptmtT/1 -> CmptmtAirTEstimdExtdComptmtT_Terminator/1
  CmptmtAirTEstimdExtdQlyFlg/1 -> CmptmtAirTEstimdExtdQlyFlg_Terminator/1
  VehMktForPmSnsrAirMtrlSnsrReq/1 -> VehMktForPmSnsrAirMtrlSnsrReq_Terminator/1
  VehMktForPmSnsrVehMktGlb/1 -> VehMktForPmSnsrVehMktGlb_Terminator/1
  IoTx_FrntBlwPwmCmd_u16_Ground/1 -> IoTx_FrntBlwPwmCmd_u16/1
  IoTx_FrntBlwFrqCmd_u16_Ground/1 -> IoTx_FrntBlwFrqCmd_u16/1
  IoRx_FrntBlwPwmFlt_u8/1 -> IoRx_FrntBlwPwmFlt_u8_Terminator/1
  IoRx_FrntBlwFrqFb_u16/1 -> IoRx_FrntBlwFrqFb_u16_Terminator/1
  IoTx_DCMot1RunDir_u8_Ground/1 -> IoTx_DCMot1RunDir_u8/1
  IoTx_DCMot2RunDir_u8_Ground/1 -> IoTx_DCMot2RunDir_u8/1
  IoTx_DCMot3RunDir_u8_Ground/1 -> IoTx_DCMot3RunDir_u8/1
  IoTx_DCMot4RunDir_u8_Ground/1 -> IoTx_DCMot4RunDir_u8/1
  IoTx_DCMot5RunDir_u8_Ground/1 -> IoTx_DCMot5RunDir_u8/1
  IoTx_DCMot6RunDir_u8_Ground/1 -> IoTx_DCMot6RunDir_u8/1
  IoTx_DCMot7RunDir_u8_Ground/1 -> IoTx_DCMot7RunDir_u8/1
  IoTx_DCMot1PwmCmd_u16_Ground/1 -> IoTx_DCMot1PwmCmd_u16/1
  IoTx_DCMot2PwmCmd_u16_Ground/1 -> IoTx_DCMot2PwmCmd_u16/1
  IoTx_DCMot3PwmCmd_u16_Ground/1 -> IoTx_DCMot3PwmCmd_u16/1
  IoTx_DCMot4PwmCmd_u16_Ground/1 -> IoTx_DCMot4PwmCmd_u16/1
  IoTx_DCMot5PwmCmd_u16_Ground/1 -> IoTx_DCMot5PwmCmd_u16/1
  IoTx_DCMot6PwmCmd_u16_Ground/1 -> IoTx_DCMot6PwmCmd_u16/1
  IoTx_DCMot7PwmCmd_u16_Ground/1 -> IoTx_DCMot7PwmCmd_u16/1
  IoTx_DCMot1FrqCmd_u16_Ground/1 -> IoTx_DCMot1FrqCmd_u16/1
  IoTx_DCMot2FrqCmd_u16_Ground/1 -> IoTx_DCMot2FrqCmd_u16/1
  IoTx_DCMot3FrqCmd_u16_Ground/1 -> IoTx_DCMot3FrqCmd_u16/1
  IoTx_DCMot4FrqCmd_u16_Ground/1 -> IoTx_DCMot4FrqCmd_u16/1
  IoTx_DCMot5FrqCmd_u16_Ground/1 -> IoTx_DCMot5FrqCmd_u16/1
  IoTx_DCMot6FrqCmd_u16_Ground/1 -> IoTx_DCMot6FrqCmd_u16/1
  IoTx_DCMot7FrqCmd_u16_Ground/1 -> IoTx_DCMot7FrqCmd_u16/1
  IoRx_DCMot1ActVoltRaw_u16/1 -> IoRx_DCMot1ActVoltRaw_u16_Terminator/1
  IoRx_DCMot2ActVoltRaw_u16/1 -> IoRx_DCMot2ActVoltRaw_u16_Terminator/1
  IoRx_DCMot3ActVoltRaw_u16/1 -> IoRx_DCMot3ActVoltRaw_u16_Terminator/1
  IoRx_DCMot4ActVoltRaw_u16/1 -> IoRx_DCMot4ActVoltRaw_u16_Terminator/1
  IoRx_DCMot5ActVoltRaw_u16/1 -> IoRx_DCMot5ActVoltRaw_u16_Terminator/1
  IoRx_DCMot6ActVoltRaw_u16/1 -> IoRx_DCMot6ActVoltRaw_u16_Terminator/1
  IoRx_DCMot7ActVoltRaw_u16/1 -> IoRx_DCMot7ActVoltRaw_u16_Terminator/1
  IoRx_DCMot1HbrFltFb_u8/1 -> IoRx_DCMot1HbrFltFb_u8_Terminator/1
  IoRx_DCMot2HbrFltFb_u8/1 -> IoRx_DCMot2HbrFltFb_u8_Terminator/1
  IoRx_DCMot3HbrFltFb_u8/1 -> IoRx_DCMot3HbrFltFb_u8_Terminator/1
  IoRx_DCMot4HbrFltFb_u8/1 -> IoRx_DCMot4HbrFltFb_u8_Terminator/1
  IoRx_DCMot5HbrFltFb_u8/1 -> IoRx_DCMot5HbrFltFb_u8_Terminator/1
  IoRx_DCMot6HbrFltFb_u8/1 -> IoRx_DCMot6HbrFltFb_u8_Terminator/1
  IoRx_DCMot7HbrFltFb_u8/1 -> IoRx_DCMot7HbrFltFb_u8_Terminator/1
  IoRx_FrntCbnTVoltRaw_u16/1 -> IoRx_FrntCbnTVoltRaw_u16_Terminator/1
  IoRx_FrntHexTVoltRaw_u16/1 -> IoRx_FrntHexTVoltRaw_u16_Terminator/1
  IoRx_FrntEvapTVoltRaw_u16/1 -> IoRx_FrntEvapTVoltRaw_u16_Terminator/1
  IoRx_FrntLeFaceTVoltRaw_u16/1 -> IoRx_FrntLeFaceTVoltRaw_u16_Terminator/1
  IoRx_FrntLeFootTVoltRaw_u16/1 -> IoRx_FrntLeFootTVoltRaw_u16_Terminator/1
  IoRx_FrntRiFaceTVoltRaw_u16/1 -> IoRx_FrntRiFaceTVoltRaw_u16_Terminator/1
  IoRx_FrntRiFootTVoltRaw_u16/1 -> IoRx_FrntRiFootTVoltRaw_u16_Terminator/1
  IoRx_ReLeFaceTVoltRaw_u16/1 -> IoRx_ReLeFaceTVoltRaw_u16_Terminator/1
  IoRx_ReLeFootTVoltRaw_u16/1 -> IoRx_ReLeFootTVoltRaw_u16_Terminator/1
  IoRx_AmbTVoltRaw_u16/1 -> IoRx_AmbTVoltRaw_u16_Terminator/1
  IoRx_EnvtAQSPwmFb_u16/1 -> IoRx_EnvtAQSPwmFb_u16_Terminator/1
  IoTx_FrntCbnTFanRly_b_Ground/1 -> IoTx_FrntCbnTFanRly_b/1
  IoRx_FrntCbnTFanRlyFlt_u8/1 -> IoRx_FrntCbnTFanRlyFlt_u8_Terminator/1
  IoTx_ClimtRly_b_Ground/1 -> IoTx_ClimtRly_b/1
  IoRx_ClimtRlyFlt_u8/1 -> IoRx_ClimtRlyFlt_u8_Terminator/1
  IoTx_ClimtPwrRly_b_Ground/1 -> IoTx_ClimtPwrRly_b/1
  IoRx_ClimtPwrRlyFlt_u8/1 -> IoRx_ClimtPwrRlyFlt_u8_Terminator/1
  IoTx_HvBattPmpPwmCmd_u16_Ground/1 -> IoTx_HvBattPmpPwmCmd_u16/1
  IoTx_HvBattPmpFrqCmd_u16_Ground/1 -> IoTx_HvBattPmpFrqCmd_u16/1
  IoRx_HvBattPmpPwmFlt_u8/1 -> IoRx_HvBattPmpPwmFlt_u8_Terminator/1
  IoTx_EldtPmpPwmCmd_u16_Ground/1 -> IoTx_EldtPmpPwmCmd_u16/1
  IoTx_EldtPmpFrqCmd_u16_Ground/1 -> IoTx_EldtPmpFrqCmd_u16/1
  IoRx_EldtPmpPwmFlt_u8/1 -> IoRx_EldtPmpPwmFlt_u8_Terminator/1
  IoTx_HeatrPmpPwmCmd_u16_Ground/1 -> IoTx_HeatrPmpPwmCmd_u16/1
  IoTx_HeatrPmpFrqCmd_u16_Ground/1 -> IoTx_HeatrPmpFrqCmd_u16/1
  IoRx_HeatrPmpPwmFlt_u8/1 -> IoRx_HeatrPmpPwmFlt_u8_Terminator/1
  IoTx_CoolgFanPwmCmd_u16_Ground/1 -> IoTx_CoolgFanPwmCmd_u16/1
  IoTx_CoolgFanFrqCmd_u16_Ground/1 -> IoTx_CoolgFanFrqCmd_u16/1
  IoRx_CoolgFanPwmFlt_u8/1 -> IoRx_CoolgFanPwmFlt_u8_Terminator/1
  IoTx_SOV1Rly_b_Ground/1 -> IoTx_SOV1Rly_b/1
  IoRx_SOV1RlyFlt_u8/1 -> IoRx_SOV1RlyFlt_u8_Terminator/1
  IoTx_SOV2Rly_b_Ground/1 -> IoTx_SOV2Rly_b/1
  IoRx_SOV2RlyFlt_u8/1 -> IoRx_SOV2RlyFlt_u8_Terminator/1
  IoTx_SOV3Rly_b_Ground/1 -> IoTx_SOV3Rly_b/1
  IoRx_SOV3RlyFlt_u8/1 -> IoRx_SOV3RlyFlt_u8_Terminator/1
  IoRx_RfgP1VoltRaw_u16/1 -> IoRx_RfgP1VoltRaw_u16_Terminator/1
  IoRx_RfgT1VoltRaw_u16/1 -> IoRx_RfgT1VoltRaw_u16_Terminator/1
  IoRx_RfgT2VoltRaw_u16/1 -> IoRx_RfgT2VoltRaw_u16_Terminator/1
  IoRx_RfgT3VoltRaw_u16/1 -> IoRx_RfgT3VoltRaw_u16_Terminator/1
  IoRx_RfgT4VoltRaw_u16/1 -> IoRx_RfgT4VoltRaw_u16_Terminator/1
  IoRx_RfgPT1PVoltRaw_u16/1 -> IoRx_RfgPT1PVoltRaw_u16_Terminator/1
  IoRx_RfgPT1TVoltRaw_u16/1 -> IoRx_RfgPT1TVoltRaw_u16_Terminator/1
  IoRx_CooltT1VoltRaw_u16/1 -> IoRx_CooltT1VoltRaw_u16_Terminator/1
  IoRx_CooltT2VoltRaw_u16/1 -> IoRx_CooltT2VoltRaw_u16_Terminator/1
  IoRx_CooltT3VoltRaw_u16/1 -> IoRx_CooltT3VoltRaw_u16_Terminator/1
  IoRx_CooltT4VoltRaw_u16/1 -> IoRx_CooltT4VoltRaw_u16_Terminator/1
  IoTx_ThermPwr1Rly_b_Ground/1 -> IoTx_ThermPwr1Rly_b/1
  IoRx_ThermPwr1RlyFlt_u8/1 -> IoRx_ThermPwr1RlyFlt_u8_Terminator/1
  IoTx_ThermPwr2Rly_b_Ground/1 -> IoTx_ThermPwr2Rly_b/1
  IoRx_ThermPwr2RlyFlt_u8/1 -> IoRx_ThermPwr2RlyFlt_u8_Terminator/1
  IoTx_ThermPwr3Rly_b_Ground/1 -> IoTx_ThermPwr3Rly_b/1
  IoRx_ThermPwr3RlyFlt_u8/1 -> IoRx_ThermPwr3RlyFlt_u8_Terminator/1
  IoTx_CoolgFanRly_b_Ground/1 -> IoTx_CoolgFanRly_b/1
  IoRx_CoolgFanRlyFlt_u8/1 -> IoRx_CoolgFanRlyFlt_u8_Terminator/1
  IoTx_PmpRly_b_Ground/1 -> IoTx_PmpRly_b/1
  IoRx_PmpRlyFlt_u8/1 -> IoRx_PmpRlyFlt_u8_Terminator/1
  RcpR_AmbTRawR/1 -> RcpR_AmbTRawR_Terminator/1
  RcpR_RfgT1RawR/1 -> RcpR_RfgT1RawR_Terminator/1
  RcpR_RfgT2RawR/1 -> RcpR_RfgT2RawR_Terminator/1
  RcpR_RfgT3RawR/1 -> RcpR_RfgT3RawR_Terminator/1
  RcpR_RfgT4RawR/1 -> RcpR_RfgT4RawR_Terminator/1
  RcpR_RfgPT1TRawR/1 -> RcpR_RfgPT1TRawR_Terminator/1
  RcpR_CooltT1RawR/1 -> RcpR_CooltT1RawR_Terminator/1
  RcpR_CooltT2RawR/1 -> RcpR_CooltT2RawR_Terminator/1
  RcpR_CooltT3RawR/1 -> RcpR_CooltT3RawR_Terminator/1
  RcpR_CooltT4RawR/1 -> RcpR_CooltT4RawR_Terminator/1
  RcpR_FrntCbnTRawR/1 -> RcpR_FrntCbnTRawR_Terminator/1
  RcpR_FrntHexTRawR/1 -> RcpR_FrntHexTRawR_Terminator/1
  RcpR_FrntEvapTRawR/1 -> RcpR_FrntEvapTRawR_Terminator/1
  RcpR_FrntLeFaceTRawR/1 -> RcpR_FrntLeFaceTRawR_Terminator/1
  RcpR_FrntLeFootTRawR/1 -> RcpR_FrntLeFootTRawR_Terminator/1
  RcpR_FrntRiFaceTRawR/1 -> RcpR_FrntRiFaceTRawR_Terminator/1
  RcpR_FrntRiFootTRawR/1 -> RcpR_FrntRiFootTRawR_Terminator/1
  RcpR_ReLeFaceTRawR/1 -> RcpR_ReLeFaceTRawR_Terminator/1
  RcpR_ReLeFootTRawR/1 -> RcpR_ReLeFootTRawR_Terminator/1
